simulink model "CloughExperimentGitHub"  (R2023a)
settings: Solver=ode45  StartTime=0.0  StopTime=t_end  FixedStep=1e-6  RelTol=relTol  AbsTol=absTol
values from neighbouring files (symbols this model uses):
  frame_rot = atan((L_beam*3/2)/(L_col/2))    [CloughExperiment.m]
  g = 9.80665    [CloughExperiment.m]    (also in Example1_CBReduction.m; GitHubVersion.m)
  gao = 1/4*chang    (= 0.3048)    [CloughExperiment.m]
  L_beam = 4*length_Convert    (= 1.2192)    [CloughExperiment.m]
  L_inplane = 6*length_Convert    (= 1.8288)    [CloughExperiment.m]
undefined symbols (not defined in the file or in its folder): aa3a, d5ee, X, Y, Z
libraries: sm_lib x165, slrealtimeloglib x29, nesl_utility x26, OxDynamicsContact x4, sharedtransform x1
(part 2 of 2)

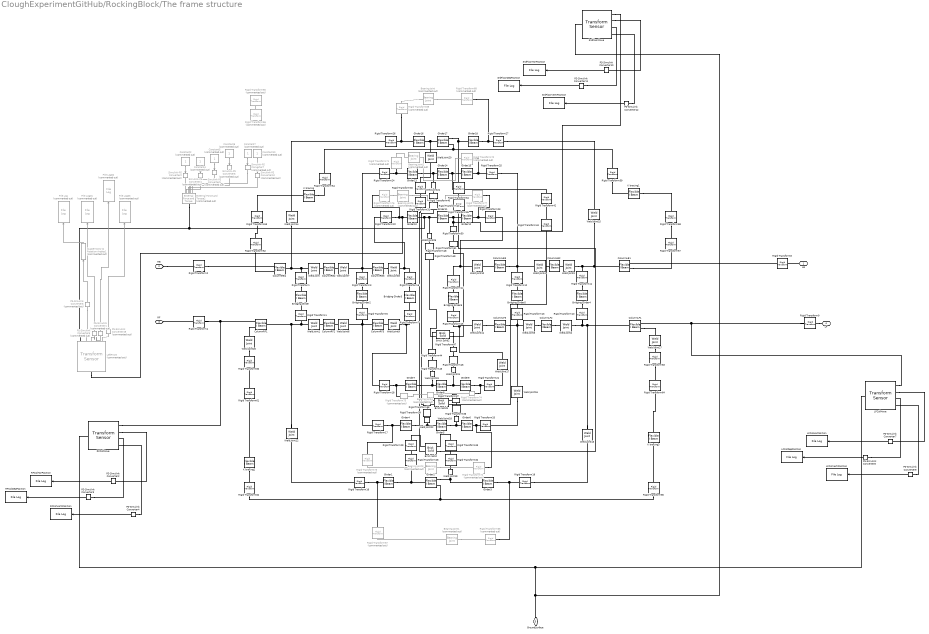
== system CloughExperimentGitHub/RockingBlock/The frame structure ==
  " LeftFront" : sm_lib/Frames and Transforms/Transform Sensor  Commented=on  MeasurementFrame=Base  RotationSequence=XYX  SenseAngle=off  SenseAxis=off  SenseQ=on  SenseR=off  SenseRotationSequence=off  SenseOmegaX=off  SenseOmegaY=off  SenseOmegaZ=off  SenseQDot=off  SenseRDot=off  SenseRotationSequenceDot=off  SenseAlphaX=off  SenseAlphaY=off  SenseAlphaZ=off  SenseQDDot=off  SenseRDDot=off  SenseX=on  SenseY=on  SenseZ=on  SenseRad=off  SenseAzim=off  SenseDist=off  SenseInc=off  SenseXDot=off  SenseYDot=off  SenseZDot=off  SenseRadDot=off  SenseAzimDot=off  SenseDistDot=off  SenseIncDot=off  SenseXDDot=off  SenseYDDot=off  SenseZDDot=off  SenseRadDDot=off  SenseAzimDDot=off  SenseDistDDot=off  SenseIncDDot=off
  3rdFloorDepPosition : slrealtimeloglib/File Log  decimation=200  inputProcessing=Elements as channels (sample based)
  3rdFloorHorPosition : slrealtimeloglib/File Log  decimation=200  inputProcessing=Elements as channels (sample based)
  3rdFloorMove : sm_lib/Frames and Transforms/Transform Sensor  MeasurementFrame=Base  RotationSequence=XYX  SenseAngle=off  SenseAxis=off  SenseQ=off  SenseR=off  SenseRotationSequence=off  SenseOmegaX=off  SenseOmegaY=off  SenseOmegaZ=off  SenseQDot=off  SenseRDot=off  SenseRotationSequenceDot=off  SenseAlphaX=off  SenseAlphaY=off  SenseAlphaZ=off  SenseQDDot=off  SenseRDDot=off  SenseX=on  SenseY=on  SenseZ=on  SenseRad=off  SenseAzim=off  SenseDist=off  SenseInc=off  SenseXDot=off  SenseYDot=off  SenseZDot=off  SenseRadDot=off  SenseAzimDot=off  SenseDistDot=off  SenseIncDot=off  SenseXDDot=off  SenseYDDot=off  SenseZDDot=off  SenseRadDDot=off  SenseAzimDDot=off  SenseDistDDot=off  SenseIncDDot=off
  3rdFloorVertiPosition : slrealtimeloglib/File Log  decimation=200  inputProcessing=Elements as channels (sample based)
  Bearing Joint{,1..5} (6 alike) : sm_lib/Joints/Bearing Joint  Commented=on  JointMode=Normal  SenseConstraintForce=off  SenseConstraintForceX=off  SenseConstraintForceY=off  SenseConstraintForceZ=off  SenseConstraintTorque=off  SenseConstraintTorqueX=off  SenseConstraintTorqueY=off  SenseConstraintTorqueZ=off  SenseTotalForce=off  SenseTotalForceX=off  SenseTotalForceY=off  SenseTotalForceZ=off  SenseTotalTorque=off  SenseTotalTorqueX=off  SenseTotalTorqueY=off  SenseTotalTorqueZ=off  CompositeWrenchDir=FollowerOnBase  CompositeWrenchFrame=BaseFrame  PzEquilibriumPosition=0  PzEquilibriumPositionUnits=m  PzSpringStiffness=0  PzSpringStiffnessUnits=N/m  PzDampingCoefficient=0  PzDampingCoefficientUnits=N/(m/s)  PzTorqueActuationMode=NoTorque  PzMotionActuationMode=ComputedMotion  PzSensePosition=off  PzSenseVelocity=off  PzSenseAcceleration=off  PzSenseTorqueForce=off  PzSenseLowerLimitTorqueForce=off  PzSenseUpperLimitTorqueForce=off  PzLowerLimitSpecify=off  PzLowerLimitBound=-1  PzLowerLimitBoundUnits=m  PzLowerLimitStiffness=1e6  PzLowerLimitStiffnessUnits=N/m  PzLowerLimitDamping=1e3  PzLowerLimitDampingUnits=N/(m/s)  PzLowerLimitTransitionRegionWidth=1e-4  PzLowerLimitTransitionRegionWidthUnits=m  PzUpperLimitSpecify=off  PzUpperLimitBound=1  PzUpperLimitBoundUnits=m  PzUpperLimitStiffness=1e6  PzUpperLimitStiffnessUnits=N/m  PzUpperLimitDamping=1e3  PzUpperLimitDampingUnits=N/(m/s)  PzUpperLimitTransitionRegionWidth=1e-4  PzUpperLimitTransitionRegionWidthUnits=m  PzPositionTargetSpecify=off  PzPositionTargetPriority=High  PzPositionTargetValue=0  PzPositionTargetValueUnits=m  PzVelocityTargetSpecify=off  PzVelocityTargetPriority=High  PzVelocityTargetValue=0  PzVelocityTargetValueUnits=m/s  RxEquilibriumPosition=0  RxEquilibriumPositionUnits=deg  RxSpringStiffness=0  RxSpringStiffnessUnits=N*m/deg  RxDampingCoefficient=0  RxDampingCoefficientUnits=N*m/(deg/s)  RxTorqueActuationMode=NoTorque  RxMotionActuationMode=ComputedMotion  RxSensePosition=off  RxSenseVelocity=off  RxSenseAcceleration=off  RxSenseTorqueForce=off  RxSenseLowerLimitTorqueForce=off  RxSenseUpperLimitTorqueForce=off  RxLowerLimitSpecify=off  RxLowerLimitBound=-90  RxLowerLimitBoundUnits=deg  RxLowerLimitStiffness=1e4  RxLowerLimitStiffnessUnits=N*m/deg  RxLowerLimitDamping=10  RxLowerLimitDampingUnits=N*m/(deg/s)  RxLowerLimitTransitionRegionWidth=0.1  RxLowerLimitTransitionRegionWidthUnits=deg  RxUpperLimitSpecify=off  RxUpperLimitBound=90  RxUpperLimitBoundUnits=deg  RxUpperLimitStiffness=1e4  RxUpperLimitStiffnessUnits=N*m/deg  RxUpperLimitDamping=10  RxUpperLimitDampingUnits=N*m/(deg/s)  RxUpperLimitTransitionRegionWidth=0.1  RxUpperLimitTransitionRegionWidthUnits=deg  RxPositionTargetSpecify=off  RxPositionTargetPriority=High  RxPositionTargetValue=0  RxPositionTargetValueUnits=deg  RxVelocityTargetSpecify=off  RxVelocityTargetPriority=High  RxVelocityTargetValue=0  RxVelocityTargetValueUnits=deg/s  RyEquilibriumPosition=0  RyEquilibriumPositionUnits=deg  RySpringStiffness=0  RySpringStiffnessUnits=N*m/deg  RyDampingCoefficient=0  RyDampingCoefficientUnits=N*m/(deg/s)  RyTorqueActuationMode=NoTorque  RyMotionActuationMode=ComputedMotion  RySensePosition=off  RySenseVelocity=off  RySenseAcceleration=off  RySenseTorqueForce=off  RySenseLowerLimitTorqueForce=off  RySenseUpperLimitTorqueForce=off  RyLowerLimitSpecify=off  RyLowerLimitBound=-90  RyLowerLimitBoundUnits=deg  RyLowerLimitStiffness=1e4  RyLowerLimitStiffnessUnits=N*m/deg  RyLowerLimitDamping=10  RyLowerLimitDampingUnits=N*m/(deg/s)  RyLowerLimitTransitionRegionWidth=0.1  RyLowerLimitTransitionRegionWidthUnits=deg  RyUpperLimitSpecify=off  RyUpperLimitBound=90  RyUpperLimitBoundUnits=deg  RyUpperLimitStiffness=1e4  RyUpperLimitStiffnessUnits=N*m/deg  RyUpperLimitDamping=10  RyUpperLimitDampingUnits=N*m/(deg/s)  RyUpperLimitTransitionRegionWidth=0.1  RyUpperLimitTransitionRegionWidthUnits=deg  RyPositionTargetSpecify=off  RyPositionTargetPriority=High  RyPositionTargetValue=0  RyPositionTargetValueUnits=deg  RyVelocityTargetSpecify=off  RyVelocityTargetPriority=High  RyVelocityTargetValue=0  RyVelocityTargetValueUnits=deg/s  RzEquilibriumPosition=0  RzEquilibriumPositionUnits=deg  RzSpringStiffness=0  RzSpringStiffnessUnits=N*m/deg  RzDampingCoefficient=0  RzDampingCoefficientUnits=N*m/(deg/s)  RzTorqueActuationMode=NoTorque  RzMotionActuationMode=ComputedMotion  RzSensePosition=off  RzSenseVelocity=off  RzSenseAcceleration=off  RzSenseTorqueForce=off  RzSenseLowerLimitTorqueForce=off  RzSenseUpperLimitTorqueForce=off  RzLowerLimitSpecify=off  RzLowerLimitBound=-90  RzLowerLimitBoundUnits=deg  RzLowerLimitStiffness=1e4  RzLowerLimitStiffnessUnits=N*m/deg  RzLowerLimitDamping=10  RzLowerLimitDampingUnits=N*m/(deg/s)  RzLowerLimitTransitionRegionWidth=0.1  RzLowerLimitTransitionRegionWidthUnits=deg  RzUpperLimitSpecify=off  RzUpperLimitBound=90  RzUpperLimitBoundUnits=deg  RzUpperLimitStiffness=1e4  RzUpperLimitStiffnessUnits=N*m/deg  RzUpperLimitDamping=10  RzUpperLimitDampingUnits=N*m/(deg/s)  RzUpperLimitTransitionRegionWidth=0.1  RzUpperLimitTransitionRegionWidthUnits=deg  RzPositionTargetSpecify=off  RzPositionTargetPriority=High  RzPositionTargetValue=0  RzPositionTargetValueUnits=deg  RzVelocityTargetSpecify=off  RzVelocityTargetPriority=High  RzVelocityTargetValue=0  RzVelocityTargetValueUnits=deg/s
  Brick Solid : sm_lib/Body Elements/Brick Solid  GraphicAmbientColor=[0.15 0.15 0.15 1.0]  BasedOnType=Density  BrickDimensions=[L_beam L_inplane gao]  BrickDimensionsUnits=m  CenterOfMass=[0 0 0]  CenterOfMassUnits=m  GraphicDiffuseColor=[0.5 0.5 0.5]  Density=rho_dw  DensityUnits=kg/m^3  DoExposeReferenceFrame=off  GraphicEmissiveColor=[0.0 0.0 0.0 1.0]  ExportEntireGeometry=off  SerializedFrames=<Frames><Frame><Id>Frame1</Id><Value><Name>F1</Name><Origin><Source>GeometricFeature</Source><FeatureName>-x +y -z point</FeatureName></Origin><PrimaryAxis><DefinedDirection>+Z</DefinedDirection><Source>ReferenceFrame</Source><SourceDirection>+Z</SourceDirection><FeatureName></FeatureName></PrimaryAxis><SecondaryAxis><DefinedDirection>+X</DefinedDirection><Source>ReferenceFrame</Source><SourceDirection>+X</SourceDirection><FeatureName></FeatureName></SecondaryAxis></Value></Frame><Frame><Id>Frame2</Id><Value><Name>F2</Name><Origin><Source>GeometricFeature</Source><FeatureName>+x +y -z point</FeatureName></Origin><PrimaryAxis><DefinedDirection>+Z</DefinedDirection><Source>ReferenceFrame</Source><SourceDirection>+Z</SourceDirection><FeatureName></FeatureName></PrimaryAxis><SecondaryAxis><DefinedDirection>+X</DefinedDirection><Source>ReferenceFrame</Source><SourceDirection>+X</SourceDirection><FeatureName></FeatureName></SecondaryAxis></Value></Frame><Frame><Id>Frame3</Id><Value><Name>F3</Name><Origin><Source>GeometricFeature</Source><FeatureName>-x -y -z point</FeatureName></Origin><PrimaryAxis><DefinedDirection>+Z</DefinedDirection><Source>ReferenceFrame</Source><SourceDirection>+Z</SourceDirection><FeatureName></FeatureName></PrimaryAxis><SecondaryAxis><DefinedDirection>+X</DefinedDirection><Source>ReferenceFrame</Source><SourceDirection>+X</SourceDirection><FeatureName></FeatureName></SecondaryAxis></Value></Frame><Frame><Id>Frame4</Id><Value><Name>F4</Name><Origin><Source>GeometricFeature</Source><FeatureName>+x -y -z point</FeatureName></Origin><PrimaryAxis><DefinedDirection>+Z</DefinedDirection><Source>ReferenceFrame</Source><SourceDirection>+Z</SourceDirection><FeatureName></FeatureName></PrimaryAxis><SecondaryAxis><DefinedDirection>+X</DefinedDirection><Source>ReferenceFrame</Source><SourceDirection>+X</SourceDirection><FeatureName></FeatureName></SecondaryAxis></Value></Frame></Frames>  MarkerShape=Sphere  MarkerSize=10  GraphicType=FromGeometry  InertiaType=CalculateFromGeometry  Mass=1  MassUnits=kg  MomentsOfInertia=[1 1 1]  MomentsOfInertiaUnits=kg*m^2  GraphicOpacity=1.0  ProductsOfInertia=[0 0 0]  ProductsOfInertiaUnits=kg*m^2  GraphicShininess=75  GraphicSpecularColor=[0.5 0.5 0.5 1.0]  GraphicVisPropType=SimpleVisualProperties
  Brick Solid1 : sm_lib/Body Elements/Brick Solid  GraphicAmbientColor=[0.15 0.15 0.15 1.0]  BasedOnType=Density  BrickDimensions=[L_beam L_inplane gao]  BrickDimensionsUnits=m  CenterOfMass=[0 0 0]  CenterOfMassUnits=m  GraphicDiffuseColor=[0.5 0.5 0.5]  Density=rho_dw  DensityUnits=kg/m^3  DoExposeReferenceFrame=off  GraphicEmissiveColor=[0.0 0.0 0.0 1.0]  ExportEntireGeometry=off  SerializedFrames=<Frames><Frame><Id>Frame1</Id><Value><Name>F1</Name><Origin><Source>GeometricFeature</Source><FeatureName>-x +y -z point</FeatureName></Origin><PrimaryAxis><DefinedDirection>+Z</DefinedDirection><Source>ReferenceFrame</Source><SourceDirection>+Z</SourceDirection><FeatureName></FeatureName></PrimaryAxis><SecondaryAxis><DefinedDirection>+X</DefinedDirection><Source>ReferenceFrame</Source><SourceDirection>+X</SourceDirection><FeatureName></FeatureName></SecondaryAxis></Value></Frame><Frame><Id>Frame2</Id><Value><Name>F2</Name><Origin><Source>GeometricFeature</Source><FeatureName>+x +y -z point</FeatureName></Origin><PrimaryAxis><DefinedDirection>+Z</DefinedDirection><Source>ReferenceFrame</Source><SourceDirection>+Z</SourceDirection><FeatureName></FeatureName></PrimaryAxis><SecondaryAxis><DefinedDirection>+X</DefinedDirection><Source>ReferenceFrame</Source><SourceDirection>+X</SourceDirection><FeatureName></FeatureName></SecondaryAxis></Value></Frame><Frame><Id>Frame3</Id><Value><Name>F3</Name><Origin><Source>GeometricFeature</Source><FeatureName>-x -y -z point</FeatureName></Origin><PrimaryAxis><DefinedDirection>+Z</DefinedDirection><Source>ReferenceFrame</Source><SourceDirection>+Z</SourceDirection><FeatureName></FeatureName></PrimaryAxis><SecondaryAxis><DefinedDirection>+X</DefinedDirection><Source>ReferenceFrame</Source><SourceDirection>+X</SourceDirection><FeatureName></FeatureName></SecondaryAxis></Value></Frame><Frame><Id>Frame4</Id><Value><Name>F4</Name><Origin><Source>GeometricFeature</Source><FeatureName>+x -y -z point</FeatureName></Origin><PrimaryAxis><DefinedDirection>+Z</DefinedDirection><Source>ReferenceFrame</Source><SourceDirection>+Z</SourceDirection><FeatureName></FeatureName></PrimaryAxis><SecondaryAxis><DefinedDirection>+X</DefinedDirection><Source>ReferenceFrame</Source><SourceDirection>+X</SourceDirection><FeatureName></FeatureName></SecondaryAxis></Value></Frame></Frames>  MarkerShape=Sphere  MarkerSize=10  GraphicType=FromGeometry  InertiaType=CalculateFromGeometry  Mass=1  MassUnits=kg  MomentsOfInertia=[1 1 1]  MomentsOfInertiaUnits=kg*m^2  GraphicOpacity=1.0  ProductsOfInertia=[0 0 0]  ProductsOfInertiaUnits=kg*m^2  GraphicShininess=75  GraphicSpecularColor=[0.5 0.5 0.5 1.0]  GraphicVisPropType=SimpleVisualProperties
  Brick Solid2 : sm_lib/Body Elements/Brick Solid  GraphicAmbientColor=[0.15 0.15 0.15 1.0]  BasedOnType=Density  BrickDimensions=[L_beam L_inplane gao]  BrickDimensionsUnits=m  CenterOfMass=[0 0 0]  CenterOfMassUnits=m  GraphicDiffuseColor=[0.5 0.5 0.5]  Density=rho_dw  DensityUnits=kg/m^3  DoExposeReferenceFrame=off  GraphicEmissiveColor=[0.0 0.0 0.0 1.0]  ExportEntireGeometry=off  SerializedFrames=<Frames><Frame><Id>Frame1</Id><Value><Name>F1</Name><Origin><Source>GeometricFeature</Source><FeatureName>-x +y -z point</FeatureName></Origin><PrimaryAxis><DefinedDirection>+Z</DefinedDirection><Source>ReferenceFrame</Source><SourceDirection>+Z</SourceDirection><FeatureName></FeatureName></PrimaryAxis><SecondaryAxis><DefinedDirection>+X</DefinedDirection><Source>ReferenceFrame</Source><SourceDirection>+X</SourceDirection><FeatureName></FeatureName></SecondaryAxis></Value></Frame><Frame><Id>Frame2</Id><Value><Name>F2</Name><Origin><Source>GeometricFeature</Source><FeatureName>+x +y -z point</FeatureName></Origin><PrimaryAxis><DefinedDirection>+Z</DefinedDirection><Source>ReferenceFrame</Source><SourceDirection>+Z</SourceDirection><FeatureName></FeatureName></PrimaryAxis><SecondaryAxis><DefinedDirection>+X</DefinedDirection><Source>ReferenceFrame</Source><SourceDirection>+X</SourceDirection><FeatureName></FeatureName></SecondaryAxis></Value></Frame><Frame><Id>Frame3</Id><Value><Name>F3</Name><Origin><Source>GeometricFeature</Source><FeatureName>-x -y -z point</FeatureName></Origin><PrimaryAxis><DefinedDirection>+Z</DefinedDirection><Source>ReferenceFrame</Source><SourceDirection>+Z</SourceDirection><FeatureName></FeatureName></PrimaryAxis><SecondaryAxis><DefinedDirection>+X</DefinedDirection><Source>ReferenceFrame</Source><SourceDirection>+X</SourceDirection><FeatureName></FeatureName></SecondaryAxis></Value></Frame><Frame><Id>Frame4</Id><Value><Name>F4</Name><Origin><Source>GeometricFeature</Source><FeatureName>+x -y -z point</FeatureName></Origin><PrimaryAxis><DefinedDirection>+Z</DefinedDirection><Source>ReferenceFrame</Source><SourceDirection>+Z</SourceDirection><FeatureName></FeatureName></PrimaryAxis><SecondaryAxis><DefinedDirection>+X</DefinedDirection><Source>ReferenceFrame</Source><SourceDirection>+X</SourceDirection><FeatureName></FeatureName></SecondaryAxis></Value></Frame></Frames>  MarkerShape=Sphere  MarkerSize=10  GraphicType=FromGeometry  InertiaType=CalculateFromGeometry  Mass=1  MassUnits=kg  MomentsOfInertia=[1 1 1]  MomentsOfInertiaUnits=kg*m^2  GraphicOpacity=1.0  ProductsOfInertia=[0 0 0]  ProductsOfInertiaUnits=kg*m^2  GraphicShininess=75  GraphicSpecularColor=[0.5 0.5 0.5 1.0]  GraphicVisPropType=SimpleVisualProperties
  Bridging Girder{,2..6} (6 alike) : sm_lib/Body Elements/Flexible Bodies/Beams/Flexible I Beam  GraphicAmbientColor=[0.15 0.15 0.15 1.0]  AxialRigidity=1  AxialRigidityUnits=Pa*m^2  BendingCentroid=[0 0]  BendingCentroidUnits=m  FlexuralRigidity=[1 1]  FlexuralRigidityUnits=Pa*m^4  BottomFlangeThickness=beam_ft  BottomFlangeThicknessUnits=m  BottomFlangeWidth=beam_fw  BottomFlangeWidthUnits=m  CenterOfMass=[0 0]  CenterOfMassUnits=m  GraphicDiffuseColor=[0.5 0.5 0.5]  CrossFlexuralRigidity=0  CrossFlexuralRigidityUnits=Pa*m^4  SerializedFrames=<Frames/>  DampingType=UniformModal  Density=rho_steel  DensityUnits=kg/m^3  DoExposeZmaxFrame=on  DoExposeZminFrame=on  GraphicEmissiveColor=[0.0 0.0 0.0 1.0]  GeometricCentroid=[0 0]  GeometricCentroidUnits=m  GraphicType=FromGeometry  EndToEndHeight=beam_depth  EndToEndHeightUnits=m  Length=L_inplane  LengthUnits=m  MassMomentOfInertiaDensity=[1 1]  MassMomentOfInertiaDensityUnits=kg*m  MassPerUnitLength=1  MassPerUnitLengthUnits=kg/m  MassProductOfInertiaDensity=0  MassProductOfInertiaDensityUnits=kg*m  ModuliType=YoungsPoissons  NumElements=1  NumRetainedModes=1  GraphicOpacity=1.0  PoissonsRatio=p_steel  ReductionType=None  ShearCenter=[0 0]  ShearCenterUnits=m  ShearModulus=26  ShearModulusUnits=GPa  GraphicShininess=75  GraphicSpecularColor=[0.5 0.5 0.5 1.0]  StiffnessAndInertiaType=CalculateFromGeometry  TopFlangeThickness=beam_ft  TopFlangeThicknessUnits=m  TopFlangeWidth=beam_fw  TopFlangeWidthUnits=m  TorsionalRigidity=1  TorsionalRigidityUnits=Pa*m^4  GraphicVisPropType=SimpleVisualProperties  WebThickness=beam_wt  WebThicknessUnits=m  YoungsModulus=E_steel  YoungsModulusUnits=Pa  ProportionalDampingAlpha=0  ProportionalDampingAlphaUnits=1/s  ProportionalDampingBeta=0.001  ProportionalDampingBetaUnits=s  UniformModalDampingRatio=uni_dr
  ColumnLB1 : sm_lib/Body Elements/Flexible Bodies/Beams/Flexible I Beam  GraphicAmbientColor=[0.15 0.15 0.15 1.0]  AxialRigidity=1  AxialRigidityUnits=Pa*m^2  BendingCentroid=[0 0]  BendingCentroidUnits=m  FlexuralRigidity=[1 1]  FlexuralRigidityUnits=Pa*m^4  BottomFlangeThickness=col_ft  BottomFlangeThicknessUnits=m  BottomFlangeWidth=col_fw  BottomFlangeWidthUnits=m  CenterOfMass=[0 0]  CenterOfMassUnits=m  GraphicDiffuseColor=[0.5 0.5 0.5]  CrossFlexuralRigidity=0  CrossFlexuralRigidityUnits=Pa*m^4  SerializedFrames=<Frames><Frame><Id>Frame1</Id><Value><Name>Middle</Name><Origin><Source>ReferenceFrame</Source><FeatureName></FeatureName></Origin><PrimaryAxis><DefinedDirection>+Z</DefinedDirection><Source>ReferenceFrame</Source><SourceDirection>+Z</SourceDirection><FeatureName></FeatureName></PrimaryAxis><SecondaryAxis><DefinedDirection>+X</DefinedDirection><Source>ReferenceFrame</Source><SourceDirection>+X</SourceDirection><FeatureName></FeatureName></SecondaryAxis></Value></Frame></Frames>  DampingType=UniformModal  Density=rho_steel  DensityUnits=kg/m^3  DoExposeZmaxFrame=on  DoExposeZminFrame=on  GraphicEmissiveColor=[0.0 0.0 0.0 1.0]  GeometricCentroid=[0 0]  GeometricCentroidUnits=m  GraphicType=FromGeometry  EndToEndHeight=col_depth  EndToEndHeightUnits=m  Length=L_col  LengthUnits=m  MassMomentOfInertiaDensity=[1 1]  MassMomentOfInertiaDensityUnits=kg*m  MassPerUnitLength=1  MassPerUnitLengthUnits=kg/m  MassProductOfInertiaDensity=0  MassProductOfInertiaDensityUnits=kg*m  ModuliType=YoungsPoissons  NumElements=2  NumRetainedModes=1  GraphicOpacity=1.0  PoissonsRatio=p_steel  ReductionType=None  ShearCenter=[0 0]  ShearCenterUnits=m  ShearModulus=26  ShearModulusUnits=GPa  GraphicShininess=75  GraphicSpecularColor=[0.5 0.5 0.5 1.0]  StiffnessAndInertiaType=CalculateFromGeometry  TopFlangeThickness=col_ft  TopFlangeThicknessUnits=m  TopFlangeWidth=col_fw  TopFlangeWidthUnits=m  TorsionalRigidity=1  TorsionalRigidityUnits=Pa*m^4  GraphicVisPropType=SimpleVisualProperties  WebThickness=col_wt  WebThicknessUnits=m  YoungsModulus=E_steel  YoungsModulusUnits=Pa  ProportionalDampingAlpha=0  ProportionalDampingAlphaUnits=1/s  ProportionalDampingBeta=0.001  ProportionalDampingBetaUnits=s  UniformModalDampingRatio=uni_dr
  ColumnLB2 : sm_lib/Body Elements/Flexible Bodies/Beams/Flexible I Beam  GraphicAmbientColor=[0.15 0.15 0.15 1.0]  AxialRigidity=1  AxialRigidityUnits=Pa*m^2  BendingCentroid=[0 0]  BendingCentroidUnits=m  FlexuralRigidity=[1 1]  FlexuralRigidityUnits=Pa*m^4  BottomFlangeThickness=col_ft  BottomFlangeThicknessUnits=m  BottomFlangeWidth=col_fw  BottomFlangeWidthUnits=m  CenterOfMass=[0 0]  CenterOfMassUnits=m  GraphicDiffuseColor=[0.5 0.5 0.5]  CrossFlexuralRigidity=0  CrossFlexuralRigidityUnits=Pa*m^4  SerializedFrames=<Frames/>  DampingType=UniformModal  Density=rho_steel  DensityUnits=kg/m^3  DoExposeZmaxFrame=on  DoExposeZminFrame=on  GraphicEmissiveColor=[0.0 0.0 0.0 1.0]  GeometricCentroid=[0 0]  GeometricCentroidUnits=m  GraphicType=FromGeometry  EndToEndHeight=col_depth  EndToEndHeightUnits=m  Length=L_col2  LengthUnits=m  MassMomentOfInertiaDensity=[1 1]  MassMomentOfInertiaDensityUnits=kg*m  MassPerUnitLength=1  MassPerUnitLengthUnits=kg/m  MassProductOfInertiaDensity=0  MassProductOfInertiaDensityUnits=kg*m  ModuliType=YoungsPoissons  NumElements=1  NumRetainedModes=1  GraphicOpacity=1.0  PoissonsRatio=p_steel  ReductionType=None  ShearCenter=[0 0]  ShearCenterUnits=m  ShearModulus=26  ShearModulusUnits=GPa  GraphicShininess=75  GraphicSpecularColor=[0.5 0.5 0.5 1.0]  StiffnessAndInertiaType=CalculateFromGeometry  TopFlangeThickness=col_ft  TopFlangeThicknessUnits=m  TopFlangeWidth=col_fw  TopFlangeWidthUnits=m  TorsionalRigidity=1  TorsionalRigidityUnits=Pa*m^4  GraphicVisPropType=SimpleVisualProperties  WebThickness=col_wt  WebThicknessUnits=m  YoungsModulus=E_steel  YoungsModulusUnits=Pa  ProportionalDampingAlpha=0  ProportionalDampingAlphaUnits=1/s  ProportionalDampingBeta=0.001  ProportionalDampingBetaUnits=s  UniformModalDampingRatio=uni_dr
  ColumnLB3 : sm_lib/Body Elements/Flexible Bodies/Beams/Flexible I Beam  GraphicAmbientColor=[0.15 0.15 0.15 1.0]  AxialRigidity=1  AxialRigidityUnits=Pa*m^2  BendingCentroid=[0 0]  BendingCentroidUnits=m  FlexuralRigidity=[1 1]  FlexuralRigidityUnits=Pa*m^4  BottomFlangeThickness=col_ft  BottomFlangeThicknessUnits=m  BottomFlangeWidth=col_fw  BottomFlangeWidthUnits=m  CenterOfMass=[0 0]  CenterOfMassUnits=m  GraphicDiffuseColor=[0.5 0.5 0.5]  CrossFlexuralRigidity=0  CrossFlexuralRigidityUnits=Pa*m^4  SerializedFrames=<Frames/>  DampingType=UniformModal  Density=rho_steel  DensityUnits=kg/m^3  DoExposeZmaxFrame=on  DoExposeZminFrame=on  GraphicEmissiveColor=[0.0 0.0 0.0 1.0]  GeometricCentroid=[0 0]  GeometricCentroidUnits=m  GraphicType=FromGeometry  EndToEndHeight=col_depth  EndToEndHeightUnits=m  Length=L_col3  LengthUnits=m  MassMomentOfInertiaDensity=[1 1]  MassMomentOfInertiaDensityUnits=kg*m  MassPerUnitLength=1  MassPerUnitLengthUnits=kg/m  MassProductOfInertiaDensity=0  MassProductOfInertiaDensityUnits=kg*m  ModuliType=YoungsPoissons  NumElements=1  NumRetainedModes=1  GraphicOpacity=1.0  PoissonsRatio=p_steel  ReductionType=None  ShearCenter=[0 0]  ShearCenterUnits=m  ShearModulus=26  ShearModulusUnits=GPa  GraphicShininess=75  GraphicSpecularColor=[0.5 0.5 0.5 1.0]  StiffnessAndInertiaType=CalculateFromGeometry  TopFlangeThickness=col_ft  TopFlangeThicknessUnits=m  TopFlangeWidth=col_fw  TopFlangeWidthUnits=m  TorsionalRigidity=1  TorsionalRigidityUnits=Pa*m^4  GraphicVisPropType=SimpleVisualProperties  WebThickness=col_wt  WebThicknessUnits=m  YoungsModulus=E_steel  YoungsModulusUnits=Pa  ProportionalDampingAlpha=0  ProportionalDampingAlphaUnits=1/s  ProportionalDampingBeta=0.001  ProportionalDampingBetaUnits=s  UniformModalDampingRatio=uni_dr
  ColumnLF1 : sm_lib/Body Elements/Flexible Bodies/Beams/Flexible I Beam  GraphicAmbientColor=[0.15 0.15 0.15 1.0]  AxialRigidity=1  AxialRigidityUnits=Pa*m^2  BendingCentroid=[0 0]  BendingCentroidUnits=m  FlexuralRigidity=[1 1]  FlexuralRigidityUnits=Pa*m^4  BottomFlangeThickness=col_ft  BottomFlangeThicknessUnits=m  BottomFlangeWidth=col_fw  BottomFlangeWidthUnits=m  CenterOfMass=[0 0]  CenterOfMassUnits=m  GraphicDiffuseColor=[0.5 0.5 0.5]  CrossFlexuralRigidity=0  CrossFlexuralRigidityUnits=Pa*m^4  SerializedFrames=<Frames><Frame><Id>Frame1</Id><Value><Name>Middle</Name><Origin><Source>ReferenceFrame</Source><FeatureName></FeatureName></Origin><PrimaryAxis><DefinedDirection>+Z</DefinedDirection><Source>ReferenceFrame</Source><SourceDirection>+Z</SourceDirection><FeatureName></FeatureName></PrimaryAxis><SecondaryAxis><DefinedDirection>+X</DefinedDirection><Source>ReferenceFrame</Source><SourceDirection>+X</SourceDirection><FeatureName></FeatureName></SecondaryAxis></Value></Frame></Frames>  DampingType=UniformModal  Density=rho_steel  DensityUnits=kg/m^3  DoExposeZmaxFrame=on  DoExposeZminFrame=on  GraphicEmissiveColor=[0.0 0.0 0.0 1.0]  GeometricCentroid=[0 0]  GeometricCentroidUnits=m  GraphicType=FromGeometry  EndToEndHeight=col_depth  EndToEndHeightUnits=m  Length=L_col  LengthUnits=m  MassMomentOfInertiaDensity=[1 1]  MassMomentOfInertiaDensityUnits=kg*m  MassPerUnitLength=1  MassPerUnitLengthUnits=kg/m  MassProductOfInertiaDensity=0  MassProductOfInertiaDensityUnits=kg*m  ModuliType=YoungsPoissons  NumElements=2  NumRetainedModes=1  GraphicOpacity=1.0  PoissonsRatio=p_steel  ReductionType=None  ShearCenter=[0 0]  ShearCenterUnits=m  ShearModulus=26  ShearModulusUnits=GPa  GraphicShininess=75  GraphicSpecularColor=[0.5 0.5 0.5 1.0]  StiffnessAndInertiaType=CalculateFromGeometry  TopFlangeThickness=col_ft  TopFlangeThicknessUnits=m  TopFlangeWidth=col_fw  TopFlangeWidthUnits=m  TorsionalRigidity=1  TorsionalRigidityUnits=Pa*m^4  GraphicVisPropType=SimpleVisualProperties  WebThickness=col_wt  WebThicknessUnits=m  YoungsModulus=E_steel  YoungsModulusUnits=Pa  ProportionalDampingAlpha=0  ProportionalDampingAlphaUnits=1/s  ProportionalDampingBeta=0.001  ProportionalDampingBetaUnits=s  UniformModalDampingRatio=uni_dr
  ColumnLF2 : sm_lib/Body Elements/Flexible Bodies/Beams/Flexible I Beam  GraphicAmbientColor=[0.15 0.15 0.15 1.0]  AxialRigidity=1  AxialRigidityUnits=Pa*m^2  BendingCentroid=[0 0]  BendingCentroidUnits=m  FlexuralRigidity=[1 1]  FlexuralRigidityUnits=Pa*m^4  BottomFlangeThickness=col_ft  BottomFlangeThicknessUnits=m  BottomFlangeWidth=col_fw  BottomFlangeWidthUnits=m  CenterOfMass=[0 0]  CenterOfMassUnits=m  GraphicDiffuseColor=[0.5 0.5 0.5]  CrossFlexuralRigidity=0  CrossFlexuralRigidityUnits=Pa*m^4  SerializedFrames=<Frames/>  DampingType=UniformModal  Density=rho_steel  DensityUnits=kg/m^3  DoExposeZmaxFrame=on  DoExposeZminFrame=on  GraphicEmissiveColor=[0.0 0.0 0.0 1.0]  GeometricCentroid=[0 0]  GeometricCentroidUnits=m  GraphicType=FromGeometry  EndToEndHeight=col_depth  EndToEndHeightUnits=m  Length=L_col2  LengthUnits=m  MassMomentOfInertiaDensity=[1 1]  MassMomentOfInertiaDensityUnits=kg*m  MassPerUnitLength=1  MassPerUnitLengthUnits=kg/m  MassProductOfInertiaDensity=0  MassProductOfInertiaDensityUnits=kg*m  ModuliType=YoungsPoissons  NumElements=1  NumRetainedModes=1  GraphicOpacity=1.0  PoissonsRatio=p_steel  ReductionType=None  ShearCenter=[0 0]  ShearCenterUnits=m  ShearModulus=26  ShearModulusUnits=GPa  GraphicShininess=75  GraphicSpecularColor=[0.5 0.5 0.5 1.0]  StiffnessAndInertiaType=CalculateFromGeometry  TopFlangeThickness=col_ft  TopFlangeThicknessUnits=m  TopFlangeWidth=col_fw  TopFlangeWidthUnits=m  TorsionalRigidity=1  TorsionalRigidityUnits=Pa*m^4  GraphicVisPropType=SimpleVisualProperties  WebThickness=col_wt  WebThicknessUnits=m  YoungsModulus=E_steel  YoungsModulusUnits=Pa  ProportionalDampingAlpha=0  ProportionalDampingAlphaUnits=1/s  ProportionalDampingBeta=0.001  ProportionalDampingBetaUnits=s  UniformModalDampingRatio=uni_dr
  ColumnLF3 : sm_lib/Body Elements/Flexible Bodies/Beams/Flexible I Beam  GraphicAmbientColor=[0.15 0.15 0.15 1.0]  AxialRigidity=1  AxialRigidityUnits=Pa*m^2  BendingCentroid=[0 0]  BendingCentroidUnits=m  FlexuralRigidity=[1 1]  FlexuralRigidityUnits=Pa*m^4  BottomFlangeThickness=col_ft  BottomFlangeThicknessUnits=m  BottomFlangeWidth=col_fw  BottomFlangeWidthUnits=m  CenterOfMass=[0 0]  CenterOfMassUnits=m  GraphicDiffuseColor=[0.5 0.5 0.5]  CrossFlexuralRigidity=0  CrossFlexuralRigidityUnits=Pa*m^4  SerializedFrames=<Frames/>  DampingType=UniformModal  Density=rho_steel  DensityUnits=kg/m^3  DoExposeZmaxFrame=on  DoExposeZminFrame=on  GraphicEmissiveColor=[0.0 0.0 0.0 1.0]  GeometricCentroid=[0 0]  GeometricCentroidUnits=m  GraphicType=FromGeometry  EndToEndHeight=col_depth  EndToEndHeightUnits=m  Length=L_col3  LengthUnits=m  MassMomentOfInertiaDensity=[1 1]  MassMomentOfInertiaDensityUnits=kg*m  MassPerUnitLength=1  MassPerUnitLengthUnits=kg/m  MassProductOfInertiaDensity=0  MassProductOfInertiaDensityUnits=kg*m  ModuliType=YoungsPoissons  NumElements=1  NumRetainedModes=1  GraphicOpacity=1.0  PoissonsRatio=p_steel  ReductionType=None  ShearCenter=[0 0]  ShearCenterUnits=m  ShearModulus=26  ShearModulusUnits=GPa  GraphicShininess=75  GraphicSpecularColor=[0.5 0.5 0.5 1.0]  StiffnessAndInertiaType=CalculateFromGeometry  TopFlangeThickness=col_ft  TopFlangeThicknessUnits=m  TopFlangeWidth=col_fw  TopFlangeWidthUnits=m  TorsionalRigidity=1  TorsionalRigidityUnits=Pa*m^4  GraphicVisPropType=SimpleVisualProperties  WebThickness=col_wt  WebThicknessUnits=m  YoungsModulus=E_steel  YoungsModulusUnits=Pa  ProportionalDampingAlpha=0  ProportionalDampingAlphaUnits=1/s  ProportionalDampingBeta=0.001  ProportionalDampingBetaUnits=s  UniformModalDampingRatio=uni_dr
  ColumnRB1 : sm_lib/Body Elements/Flexible Bodies/Beams/Flexible I Beam  GraphicAmbientColor=[0.15 0.15 0.15 1.0]  AxialRigidity=1  AxialRigidityUnits=Pa*m^2  BendingCentroid=[0 0]  BendingCentroidUnits=m  FlexuralRigidity=[1 1]  FlexuralRigidityUnits=Pa*m^4  BottomFlangeThickness=col_ft  BottomFlangeThicknessUnits=m  BottomFlangeWidth=col_fw  BottomFlangeWidthUnits=m  CenterOfMass=[0 0]  CenterOfMassUnits=m  GraphicDiffuseColor=[0.5 0.5 0.5]  CrossFlexuralRigidity=0  CrossFlexuralRigidityUnits=Pa*m^4  SerializedFrames=<Frames><Frame><Id>Frame1</Id><Value><Name>Middle</Name><Origin><Source>ReferenceFrame</Source><FeatureName></FeatureName></Origin><PrimaryAxis><DefinedDirection>+Z</DefinedDirection><Source>ReferenceFrame</Source><SourceDirection>+Z</SourceDirection><FeatureName></FeatureName></PrimaryAxis><SecondaryAxis><DefinedDirection>+X</DefinedDirection><Source>ReferenceFrame</Source><SourceDirection>+X</SourceDirection><FeatureName></FeatureName></SecondaryAxis></Value></Frame></Frames>  DampingType=UniformModal  Density=rho_steel  DensityUnits=kg/m^3  DoExposeZmaxFrame=on  DoExposeZminFrame=on  GraphicEmissiveColor=[0.0 0.0 0.0 1.0]  GeometricCentroid=[0 0]  GeometricCentroidUnits=m  GraphicType=FromGeometry  EndToEndHeight=col_depth  EndToEndHeightUnits=m  Length=L_col  LengthUnits=m  MassMomentOfInertiaDensity=[1 1]  MassMomentOfInertiaDensityUnits=kg*m  MassPerUnitLength=1  MassPerUnitLengthUnits=kg/m  MassProductOfInertiaDensity=0  MassProductOfInertiaDensityUnits=kg*m  ModuliType=YoungsPoissons  NumElements=2  NumRetainedModes=1  GraphicOpacity=1.0  PoissonsRatio=p_steel  ReductionType=None  ShearCenter=[0 0]  ShearCenterUnits=m  ShearModulus=26  ShearModulusUnits=GPa  GraphicShininess=75  GraphicSpecularColor=[0.5 0.5 0.5 1.0]  StiffnessAndInertiaType=CalculateFromGeometry  TopFlangeThickness=col_ft  TopFlangeThicknessUnits=m  TopFlangeWidth=col_fw  TopFlangeWidthUnits=m  TorsionalRigidity=1  TorsionalRigidityUnits=Pa*m^4  GraphicVisPropType=SimpleVisualProperties  WebThickness=col_wt  WebThicknessUnits=m  YoungsModulus=E_steel  YoungsModulusUnits=Pa  ProportionalDampingAlpha=0  ProportionalDampingAlphaUnits=1/s  ProportionalDampingBeta=0.001  ProportionalDampingBetaUnits=s  UniformModalDampingRatio=uni_dr
  ColumnRB2 : sm_lib/Body Elements/Flexible Bodies/Beams/Flexible I Beam  GraphicAmbientColor=[0.15 0.15 0.15 1.0]  AxialRigidity=1  AxialRigidityUnits=Pa*m^2  BendingCentroid=[0 0]  BendingCentroidUnits=m  FlexuralRigidity=[1 1]  FlexuralRigidityUnits=Pa*m^4  BottomFlangeThickness=col_ft  BottomFlangeThicknessUnits=m  BottomFlangeWidth=col_fw  BottomFlangeWidthUnits=m  CenterOfMass=[0 0]  CenterOfMassUnits=m  GraphicDiffuseColor=[0.5 0.5 0.5]  CrossFlexuralRigidity=0  CrossFlexuralRigidityUnits=Pa*m^4  SerializedFrames=<Frames/>  DampingType=UniformModal  Density=rho_steel  DensityUnits=kg/m^3  DoExposeZmaxFrame=on  DoExposeZminFrame=on  GraphicEmissiveColor=[0.0 0.0 0.0 1.0]  GeometricCentroid=[0 0]  GeometricCentroidUnits=m  GraphicType=FromGeometry  EndToEndHeight=col_depth  EndToEndHeightUnits=m  Length=L_col2  LengthUnits=m  MassMomentOfInertiaDensity=[1 1]  MassMomentOfInertiaDensityUnits=kg*m  MassPerUnitLength=1  MassPerUnitLengthUnits=kg/m  MassProductOfInertiaDensity=0  MassProductOfInertiaDensityUnits=kg*m  ModuliType=YoungsPoissons  NumElements=1  NumRetainedModes=1  GraphicOpacity=1.0  PoissonsRatio=p_steel  ReductionType=None  ShearCenter=[0 0]  ShearCenterUnits=m  ShearModulus=26  ShearModulusUnits=GPa  GraphicShininess=75  GraphicSpecularColor=[0.5 0.5 0.5 1.0]  StiffnessAndInertiaType=CalculateFromGeometry  TopFlangeThickness=col_ft  TopFlangeThicknessUnits=m  TopFlangeWidth=col_fw  TopFlangeWidthUnits=m  TorsionalRigidity=1  TorsionalRigidityUnits=Pa*m^4  GraphicVisPropType=SimpleVisualProperties  WebThickness=col_wt  WebThicknessUnits=m  YoungsModulus=E_steel  YoungsModulusUnits=Pa  ProportionalDampingAlpha=0  ProportionalDampingAlphaUnits=1/s  ProportionalDampingBeta=0.001  ProportionalDampingBetaUnits=s  UniformModalDampingRatio=uni_dr
  ColumnRB3 : sm_lib/Body Elements/Flexible Bodies/Beams/Flexible I Beam  GraphicAmbientColor=[0.15 0.15 0.15 1.0]  AxialRigidity=1  AxialRigidityUnits=Pa*m^2  BendingCentroid=[0 0]  BendingCentroidUnits=m  FlexuralRigidity=[1 1]  FlexuralRigidityUnits=Pa*m^4  BottomFlangeThickness=col_ft  BottomFlangeThicknessUnits=m  BottomFlangeWidth=col_fw  BottomFlangeWidthUnits=m  CenterOfMass=[0 0]  CenterOfMassUnits=m  GraphicDiffuseColor=[0.5 0.5 0.5]  CrossFlexuralRigidity=0  CrossFlexuralRigidityUnits=Pa*m^4  SerializedFrames=<Frames/>  DampingType=UniformModal  Density=rho_steel  DensityUnits=kg/m^3  DoExposeZmaxFrame=on  DoExposeZminFrame=on  GraphicEmissiveColor=[0.0 0.0 0.0 1.0]  GeometricCentroid=[0 0]  GeometricCentroidUnits=m  GraphicType=FromGeometry  EndToEndHeight=col_depth  EndToEndHeightUnits=m  Length=L_col3  LengthUnits=m  MassMomentOfInertiaDensity=[1 1]  MassMomentOfInertiaDensityUnits=kg*m  MassPerUnitLength=1  MassPerUnitLengthUnits=kg/m  MassProductOfInertiaDensity=0  MassProductOfInertiaDensityUnits=kg*m  ModuliType=YoungsPoissons  NumElements=1  NumRetainedModes=1  GraphicOpacity=1.0  PoissonsRatio=p_steel  ReductionType=None  ShearCenter=[0 0]  ShearCenterUnits=m  ShearModulus=26  ShearModulusUnits=GPa  GraphicShininess=75  GraphicSpecularColor=[0.5 0.5 0.5 1.0]  StiffnessAndInertiaType=CalculateFromGeometry  TopFlangeThickness=col_ft  TopFlangeThicknessUnits=m  TopFlangeWidth=col_fw  TopFlangeWidthUnits=m  TorsionalRigidity=1  TorsionalRigidityUnits=Pa*m^4  GraphicVisPropType=SimpleVisualProperties  WebThickness=col_wt  WebThicknessUnits=m  YoungsModulus=E_steel  YoungsModulusUnits=Pa  ProportionalDampingAlpha=0  ProportionalDampingAlphaUnits=1/s  ProportionalDampingBeta=0.001  ProportionalDampingBetaUnits=s  UniformModalDampingRatio=uni_dr
  ColumnRF1 : sm_lib/Body Elements/Flexible Bodies/Beams/Flexible I Beam  GraphicAmbientColor=[0.15 0.15 0.15 1.0]  AxialRigidity=1  AxialRigidityUnits=Pa*m^2  BendingCentroid=[0 0]  BendingCentroidUnits=m  FlexuralRigidity=[1 1]  FlexuralRigidityUnits=Pa*m^4  BottomFlangeThickness=col_ft  BottomFlangeThicknessUnits=m  BottomFlangeWidth=col_fw  BottomFlangeWidthUnits=m  CenterOfMass=[0 0]  CenterOfMassUnits=m  GraphicDiffuseColor=[0.5 0.5 0.5]  CrossFlexuralRigidity=0  CrossFlexuralRigidityUnits=Pa*m^4  SerializedFrames=<Frames><Frame><Id>Frame1</Id><Value><Name>Middle</Name><Origin><Source>ReferenceFrame</Source><FeatureName></FeatureName></Origin><PrimaryAxis><DefinedDirection>+Z</DefinedDirection><Source>ReferenceFrame</Source><SourceDirection>+Z</SourceDirection><FeatureName></FeatureName></PrimaryAxis><SecondaryAxis><DefinedDirection>+X</DefinedDirection><Source>ReferenceFrame</Source><SourceDirection>+X</SourceDirection><FeatureName></FeatureName></SecondaryAxis></Value></Frame></Frames>  DampingType=UniformModal  Density=rho_steel  DensityUnits=kg/m^3  DoExposeZmaxFrame=on  DoExposeZminFrame=on  GraphicEmissiveColor=[0.0 0.0 0.0 1.0]  GeometricCentroid=[0 0]  GeometricCentroidUnits=m  GraphicType=FromGeometry  EndToEndHeight=col_depth  EndToEndHeightUnits=m  Length=L_col  LengthUnits=m  MassMomentOfInertiaDensity=[1 1]  MassMomentOfInertiaDensityUnits=kg*m  MassPerUnitLength=1  MassPerUnitLengthUnits=kg/m  MassProductOfInertiaDensity=0  MassProductOfInertiaDensityUnits=kg*m  ModuliType=YoungsPoissons  NumElements=2  NumRetainedModes=1  GraphicOpacity=1.0  PoissonsRatio=p_steel  ReductionType=None  ShearCenter=[0 0]  ShearCenterUnits=m  ShearModulus=26  ShearModulusUnits=GPa  GraphicShininess=75  GraphicSpecularColor=[0.5 0.5 0.5 1.0]  StiffnessAndInertiaType=CalculateFromGeometry  TopFlangeThickness=col_ft  TopFlangeThicknessUnits=m  TopFlangeWidth=col_fw  TopFlangeWidthUnits=m  TorsionalRigidity=1  TorsionalRigidityUnits=Pa*m^4  GraphicVisPropType=SimpleVisualProperties  WebThickness=col_wt  WebThicknessUnits=m  YoungsModulus=E_steel  YoungsModulusUnits=Pa  ProportionalDampingAlpha=0  ProportionalDampingAlphaUnits=1/s  ProportionalDampingBeta=0.001  ProportionalDampingBetaUnits=s  UniformModalDampingRatio=uni_dr
  ColumnRF2 : sm_lib/Body Elements/Flexible Bodies/Beams/Flexible I Beam  GraphicAmbientColor=[0.15 0.15 0.15 1.0]  AxialRigidity=1  AxialRigidityUnits=Pa*m^2  BendingCentroid=[0 0]  BendingCentroidUnits=m  FlexuralRigidity=[1 1]  FlexuralRigidityUnits=Pa*m^4  BottomFlangeThickness=col_ft  BottomFlangeThicknessUnits=m  BottomFlangeWidth=col_fw  BottomFlangeWidthUnits=m  CenterOfMass=[0 0]  CenterOfMassUnits=m  GraphicDiffuseColor=[0.5 0.5 0.5]  CrossFlexuralRigidity=0  CrossFlexuralRigidityUnits=Pa*m^4  SerializedFrames=<Frames/>  DampingType=UniformModal  Density=rho_steel  DensityUnits=kg/m^3  DoExposeZmaxFrame=on  DoExposeZminFrame=on  GraphicEmissiveColor=[0.0 0.0 0.0 1.0]  GeometricCentroid=[0 0]  GeometricCentroidUnits=m  GraphicType=FromGeometry  EndToEndHeight=col_depth  EndToEndHeightUnits=m  Length=L_col2  LengthUnits=m  MassMomentOfInertiaDensity=[1 1]  MassMomentOfInertiaDensityUnits=kg*m  MassPerUnitLength=1  MassPerUnitLengthUnits=kg/m  MassProductOfInertiaDensity=0  MassProductOfInertiaDensityUnits=kg*m  ModuliType=YoungsPoissons  NumElements=1  NumRetainedModes=1  GraphicOpacity=1.0  PoissonsRatio=p_steel  ReductionType=None  ShearCenter=[0 0]  ShearCenterUnits=m  ShearModulus=26  ShearModulusUnits=GPa  GraphicShininess=75  GraphicSpecularColor=[0.5 0.5 0.5 1.0]  StiffnessAndInertiaType=CalculateFromGeometry  TopFlangeThickness=col_ft  TopFlangeThicknessUnits=m  TopFlangeWidth=col_fw  TopFlangeWidthUnits=m  TorsionalRigidity=1  TorsionalRigidityUnits=Pa*m^4  GraphicVisPropType=SimpleVisualProperties  WebThickness=col_wt  WebThicknessUnits=m  YoungsModulus=E_steel  YoungsModulusUnits=Pa  ProportionalDampingAlpha=0  ProportionalDampingAlphaUnits=1/s  ProportionalDampingBeta=0.001  ProportionalDampingBetaUnits=s  UniformModalDampingRatio=uni_dr
  ColumnRF3 : sm_lib/Body Elements/Flexible Bodies/Beams/Flexible I Beam  GraphicAmbientColor=[0.15 0.15 0.15 1.0]  AxialRigidity=1  AxialRigidityUnits=Pa*m^2  BendingCentroid=[0 0]  BendingCentroidUnits=m  FlexuralRigidity=[1 1]  FlexuralRigidityUnits=Pa*m^4  BottomFlangeThickness=col_ft  BottomFlangeThicknessUnits=m  BottomFlangeWidth=col_fw  BottomFlangeWidthUnits=m  CenterOfMass=[0 0]  CenterOfMassUnits=m  GraphicDiffuseColor=[0.5 0.5 0.5]  CrossFlexuralRigidity=0  CrossFlexuralRigidityUnits=Pa*m^4  SerializedFrames=<Frames/>  DampingType=UniformModal  Density=rho_steel  DensityUnits=kg/m^3  DoExposeZmaxFrame=on  DoExposeZminFrame=on  GraphicEmissiveColor=[0.0 0.0 0.0 1.0]  GeometricCentroid=[0 0]  GeometricCentroidUnits=m  GraphicType=FromGeometry  EndToEndHeight=col_depth  EndToEndHeightUnits=m  Length=L_col3  LengthUnits=m  MassMomentOfInertiaDensity=[1 1]  MassMomentOfInertiaDensityUnits=kg*m  MassPerUnitLength=1  MassPerUnitLengthUnits=kg/m  MassProductOfInertiaDensity=0  MassProductOfInertiaDensityUnits=kg*m  ModuliType=YoungsPoissons  NumElements=1  NumRetainedModes=1  GraphicOpacity=1.0  PoissonsRatio=p_steel  ReductionType=None  ShearCenter=[0 0]  ShearCenterUnits=m  ShearModulus=26  ShearModulusUnits=GPa  GraphicShininess=75  GraphicSpecularColor=[0.5 0.5 0.5 1.0]  StiffnessAndInertiaType=CalculateFromGeometry  TopFlangeThickness=col_ft  TopFlangeThicknessUnits=m  TopFlangeWidth=col_fw  TopFlangeWidthUnits=m  TorsionalRigidity=1  TorsionalRigidityUnits=Pa*m^4  GraphicVisPropType=SimpleVisualProperties  WebThickness=col_wt  WebThicknessUnits=m  YoungsModulus=E_steel  YoungsModulusUnits=Pa  ProportionalDampingAlpha=0  ProportionalDampingAlphaUnits=1/s  ProportionalDampingBeta=0.001  ProportionalDampingBetaUnits=s  UniformModalDampingRatio=uni_dr
  Constant{2,4..7,10} (6 alike) : Constant  Commented=on
  External Force and Torque2 : sm_lib/Forces and Torques/External Force and Torque  Commented=on  ForceResolutionFrame=AttachedFrame  EnableForceX=on  EnableForceY=on  EnableForceZ=on  EnableForce=off  TorqueResolutionFrame=AttachedFrame  EnableTorqueX=on  EnableTorqueY=on  EnableTorqueZ=on  EnableTorque=off
  File Log : slrealtimeloglib/File Log  Commented=on  decimation=50  inputProcessing=Elements as channels (sample based)
  File Log01 : slrealtimeloglib/File Log  Commented=on  decimation=50  inputProcessing=Elements as channels (sample based)
  File Log02 : slrealtimeloglib/File Log  Commented=on  decimation=50  inputProcessing=Elements as channels (sample based)
  File Log03 : slrealtimeloglib/File Log  Commented=on  decimation=50  inputProcessing=Elements as channels (sample based)
  Girder{1,3..16,18} (16 alike) : sm_lib/Body Elements/Flexible Bodies/Beams/Flexible I Beam  GraphicAmbientColor=[0.15 0.15 0.15 1.0]  AxialRigidity=1  AxialRigidityUnits=Pa*m^2  BendingCentroid=[0 0]  BendingCentroidUnits=m  FlexuralRigidity=[1 1]  FlexuralRigidityUnits=Pa*m^4  BottomFlangeThickness=beam_ft  BottomFlangeThicknessUnits=m  BottomFlangeWidth=beam_fw  BottomFlangeWidthUnits=m  CenterOfMass=[0 0]  CenterOfMassUnits=m  GraphicDiffuseColor=[0.5 0.5 0.5]  CrossFlexuralRigidity=0  CrossFlexuralRigidityUnits=Pa*m^4  SerializedFrames=<Frames/>  DampingType=UniformModal  Density=rho_steel  DensityUnits=kg/m^3  DoExposeZmaxFrame=on  DoExposeZminFrame=on  GraphicEmissiveColor=[0.0 0.0 0.0 1.0]  GeometricCentroid=[0 0]  GeometricCentroidUnits=m  GraphicType=FromGeometry  EndToEndHeight=beam_depth  EndToEndHeightUnits=m  Length=L_beam  LengthUnits=m  MassMomentOfInertiaDensity=[1 1]  MassMomentOfInertiaDensityUnits=kg*m  MassPerUnitLength=1  MassPerUnitLengthUnits=kg/m  MassProductOfInertiaDensity=0  MassProductOfInertiaDensityUnits=kg*m  ModuliType=YoungsPoissons  NumElements=1  NumRetainedModes=1  GraphicOpacity=1.0  PoissonsRatio=p_steel  ReductionType=None  ShearCenter=[0 0]  ShearCenterUnits=m  ShearModulus=26  ShearModulusUnits=GPa  GraphicShininess=75  GraphicSpecularColor=[0.5 0.5 0.5 1.0]  StiffnessAndInertiaType=CalculateFromGeometry  TopFlangeThickness=beam_ft  TopFlangeThicknessUnits=m  TopFlangeWidth=beam_fw  TopFlangeWidthUnits=m  TorsionalRigidity=1  TorsionalRigidityUnits=Pa*m^4  GraphicVisPropType=SimpleVisualProperties  WebThickness=beam_wt  WebThicknessUnits=m  YoungsModulus=E_steel  YoungsModulusUnits=Pa  ProportionalDampingAlpha=0  ProportionalDampingAlphaUnits=1/s  ProportionalDampingBeta=0.001  ProportionalDampingBetaUnits=s  UniformModalDampingRatio=uni_dr
  Girder17 : sm_lib/Body Elements/Flexible Bodies/Beams/Flexible I Beam  GraphicAmbientColor=[0.15 0.15 0.15 1.0]  AxialRigidity=1  AxialRigidityUnits=Pa*m^2  BendingCentroid=[0 0]  BendingCentroidUnits=m  FlexuralRigidity=[1 1]  FlexuralRigidityUnits=Pa*m^4  BottomFlangeThickness=beam_ft  BottomFlangeThicknessUnits=m  BottomFlangeWidth=beam_fw  BottomFlangeWidthUnits=m  CenterOfMass=[0 0]  CenterOfMassUnits=m  GraphicDiffuseColor=[0.5 0.5 0.5]  CrossFlexuralRigidity=0  CrossFlexuralRigidityUnits=Pa*m^4  SerializedFrames=<Frames><Frame><Id>Frame1</Id><Value><Name>Middle</Name><Origin><Source>ReferenceFrame</Source><FeatureName></FeatureName></Origin><PrimaryAxis><DefinedDirection>+Z</DefinedDirection><Source>ReferenceFrame</Source><SourceDirection>+Z</SourceDirection><FeatureName></FeatureName></PrimaryAxis><SecondaryAxis><DefinedDirection>+X</DefinedDirection><Source>ReferenceFrame</Source><SourceDirection>+X</SourceDirection><FeatureName></FeatureName></SecondaryAxis></Value></Frame></Frames>  DampingType=UniformModal  Density=rho_steel  DensityUnits=kg/m^3  DoExposeZmaxFrame=on  DoExposeZminFrame=on  GraphicEmissiveColor=[0.0 0.0 0.0 1.0]  GeometricCentroid=[0 0]  GeometricCentroidUnits=m  GraphicType=FromGeometry  EndToEndHeight=beam_depth  EndToEndHeightUnits=m  Length=L_beam  LengthUnits=m  MassMomentOfInertiaDensity=[1 1]  MassMomentOfInertiaDensityUnits=kg*m  MassPerUnitLength=1  MassPerUnitLengthUnits=kg/m  MassProductOfInertiaDensity=0  MassProductOfInertiaDensityUnits=kg*m  ModuliType=YoungsPoissons  NumElements=2  NumRetainedModes=1  GraphicOpacity=1.0  PoissonsRatio=p_steel  ReductionType=None  ShearCenter=[0 0]  ShearCenterUnits=m  ShearModulus=26  ShearModulusUnits=GPa  GraphicShininess=75  GraphicSpecularColor=[0.5 0.5 0.5 1.0]  StiffnessAndInertiaType=CalculateFromGeometry  TopFlangeThickness=beam_ft  TopFlangeThicknessUnits=m  TopFlangeWidth=beam_fw  TopFlangeWidthUnits=m  TorsionalRigidity=1  TorsionalRigidityUnits=Pa*m^4  GraphicVisPropType=SimpleVisualProperties  WebThickness=beam_wt  WebThicknessUnits=m  YoungsModulus=E_steel  YoungsModulusUnits=Pa  ProportionalDampingAlpha=0  ProportionalDampingAlphaUnits=1/s  ProportionalDampingBeta=0.001  ProportionalDampingBetaUnits=s  UniformModalDampingRatio=uni_dr
  Girder2 : sm_lib/Body Elements/Flexible Bodies/Beams/Flexible I Beam  GraphicAmbientColor=[0.15 0.15 0.15 1.0]  AxialRigidity=1  AxialRigidityUnits=Pa*m^2  BendingCentroid=[0 0]  BendingCentroidUnits=m  FlexuralRigidity=[1 1]  FlexuralRigidityUnits=Pa*m^4  BottomFlangeThickness=beam_ft  BottomFlangeThicknessUnits=m  BottomFlangeWidth=beam_fw  BottomFlangeWidthUnits=m  CenterOfMass=[0 0]  CenterOfMassUnits=m  GraphicDiffuseColor=[0.5 0.5 0.5]  CrossFlexuralRigidity=0  CrossFlexuralRigidityUnits=Pa*m^4  SerializedFrames=<Frames><Frame><Id>Frame1</Id><Value><Name>Middle</Name><Origin><Source>ReferenceFrame</Source><FeatureName></FeatureName></Origin><PrimaryAxis><DefinedDirection>+Z</DefinedDirection><Source>ReferenceFrame</Source><SourceDirection>+Z</SourceDirection><FeatureName></FeatureName></PrimaryAxis><SecondaryAxis><DefinedDirection>+X</DefinedDirection><Source>ReferenceFrame</Source><SourceDirection>+X</SourceDirection><FeatureName></FeatureName></SecondaryAxis></Value></Frame></Frames>  DampingType=UniformModal  Density=rho_steel  DensityUnits=kg/m^3  DoExposeZmaxFrame=on  DoExposeZminFrame=on  GraphicEmissiveColor=[0.0 0.0 0.0 1.0]  GeometricCentroid=[0 0]  GeometricCentroidUnits=m  GraphicType=FromGeometry  EndToEndHeight=beam_depth  EndToEndHeightUnits=m  Length=L_beam  LengthUnits=m  MassMomentOfInertiaDensity=[1 1]  MassMomentOfInertiaDensityUnits=kg*m  MassPerUnitLength=1  MassPerUnitLengthUnits=kg/m  MassProductOfInertiaDensity=0  MassProductOfInertiaDensityUnits=kg*m  ModuliType=YoungsPoissons  NumElements=2  NumRetainedModes=1  GraphicOpacity=1.0  PoissonsRatio=p_steel  ReductionType=None  ShearCenter=[0 0]  ShearCenterUnits=m  ShearModulus=26  ShearModulusUnits=GPa  GraphicShininess=75  GraphicSpecularColor=[0.5 0.5 0.5 1.0]  StiffnessAndInertiaType=CalculateFromGeometry  TopFlangeThickness=beam_ft  TopFlangeThicknessUnits=m  TopFlangeWidth=beam_fw  TopFlangeWidthUnits=m  TorsionalRigidity=1  TorsionalRigidityUnits=Pa*m^4  GraphicVisPropType=SimpleVisualProperties  WebThickness=beam_wt  WebThicknessUnits=m  YoungsModulus=E_steel  YoungsModulusUnits=Pa  ProportionalDampingAlpha=0  ProportionalDampingAlphaUnits=1/s  ProportionalDampingBeta=0.001  ProportionalDampingBetaUnits=s  UniformModalDampingRatio=uni_dr
  K bracing{,1..3} (4 alike) : sm_lib/Body Elements/Flexible Bodies/Beams/Flexible I Beam  GraphicAmbientColor=[0.15 0.15 0.15 1.0]  AxialRigidity=1  AxialRigidityUnits=Pa*m^2  BendingCentroid=[0 0]  BendingCentroidUnits=m  FlexuralRigidity=[1 1]  FlexuralRigidityUnits=Pa*m^4  BottomFlangeThickness=beam_ft  BottomFlangeThicknessUnits=m  BottomFlangeWidth=beam_fw  BottomFlangeWidthUnits=m  CenterOfMass=[0 0]  CenterOfMassUnits=m  GraphicDiffuseColor=[0.5 0.5 0.5]  CrossFlexuralRigidity=0  CrossFlexuralRigidityUnits=Pa*m^4  SerializedFrames=<Frames/>  DampingType=UniformModal  Density=rho_steel  DensityUnits=kg/m^3  DoExposeZmaxFrame=on  DoExposeZminFrame=on  GraphicEmissiveColor=[0.0 0.0 0.0 1.0]  GeometricCentroid=[0 0]  GeometricCentroidUnits=m  GraphicType=FromGeometry  EndToEndHeight=beam_depth  EndToEndHeightUnits=m  Length=L_brace  LengthUnits=m  MassMomentOfInertiaDensity=[1 1]  MassMomentOfInertiaDensityUnits=kg*m  MassPerUnitLength=1  MassPerUnitLengthUnits=kg/m  MassProductOfInertiaDensity=0  MassProductOfInertiaDensityUnits=kg*m  ModuliType=YoungsPoissons  NumElements=1  NumRetainedModes=1  GraphicOpacity=1.0  PoissonsRatio=p_steel  ReductionType=None  ShearCenter=[0 0]  ShearCenterUnits=m  ShearModulus=26  ShearModulusUnits=GPa  GraphicShininess=75  GraphicSpecularColor=[0.5 0.5 0.5 1.0]  StiffnessAndInertiaType=CalculateFromGeometry  TopFlangeThickness=beam_ft  TopFlangeThicknessUnits=m  TopFlangeWidth=beam_fw  TopFlangeWidthUnits=m  TorsionalRigidity=1  TorsionalRigidityUnits=Pa*m^4  GraphicVisPropType=SimpleVisualProperties  WebThickness=beam_wt  WebThicknessUnits=m  YoungsModulus=E_steel  YoungsModulusUnits=Pa  ProportionalDampingAlpha=0  ProportionalDampingAlphaUnits=1/s  ProportionalDampingBeta=0.001  ProportionalDampingBetaUnits=s  UniformModalDampingRatio=uni_dr
  LFColDepPosition : slrealtimeloglib/File Log  decimation=200  inputProcessing=Elements as channels (sample based)
  LFColHorPosition : slrealtimeloglib/File Log  decimation=200  inputProcessing=Elements as channels (sample based)
  LFColMove : sm_lib/Frames and Transforms/Transform Sensor  MeasurementFrame=Base  RotationSequence=XYX  SenseAngle=off  SenseAxis=off  SenseQ=off  SenseR=off  SenseRotationSequence=off  SenseOmegaX=off  SenseOmegaY=off  SenseOmegaZ=off  SenseQDot=off  SenseRDot=off  SenseRotationSequenceDot=off  SenseAlphaX=off  SenseAlphaY=off  SenseAlphaZ=off  SenseQDDot=off  SenseRDDot=off  SenseX=on  SenseY=on  SenseZ=on  SenseRad=off  SenseAzim=off  SenseDist=off  SenseInc=off  SenseXDot=off  SenseYDot=off  SenseZDot=off  SenseRadDot=off  SenseAzimDot=off  SenseDistDot=off  SenseIncDot=off  SenseXDDot=off  SenseYDDot=off  SenseZDDot=off  SenseRadDDot=off  SenseAzimDDot=off  SenseDistDDot=off  SenseIncDDot=off
  LFColVertiPosition : slrealtimeloglib/File Log  decimation=200  inputProcessing=Elements as channels (sample based)
  PS-Simulink Converter{1,5..6,19} (4 alike) : nesl_utility/PS-Simulink Converter  Commented=on  PhysicalDomain=network_engine_domain  SubClassName=ps_output  LeftPortType=input  RightPortType=output  PseudoPeriodic=off  Frequencies=[]  VectorFormat=1-D array  Unit=inherit  AffineConversion=off
  PS-Simulink Converter{2..4,7..12} (9 alike) : nesl_utility/PS-Simulink Converter  PhysicalDomain=network_engine_domain  SubClassName=ps_output  LeftPortType=input  RightPortType=output  PseudoPeriodic=off  Frequencies=[]  VectorFormat=1-D array  Unit=inherit  AffineConversion=off
  Quaternions to Rotation Angles1 : sharedtransform/Quaternions to Rotation Angles  Commented=on  rotationOrder=XYZ  aMode=aMode
  RFColDepPosition : slrealtimeloglib/File Log  decimation=200  inputProcessing=Elements as channels (sample based)
  RFColHorPosition : slrealtimeloglib/File Log  decimation=200  inputProcessing=Elements as channels (sample based)
  RFColMove : sm_lib/Frames and Transforms/Transform Sensor  MeasurementFrame=Base  RotationSequence=XYX  SenseAngle=off  SenseAxis=off  SenseQ=off  SenseR=off  SenseRotationSequence=off  SenseOmegaX=off  SenseOmegaY=off  SenseOmegaZ=off  SenseQDot=off  SenseRDot=off  SenseRotationSequenceDot=off  SenseAlphaX=off  SenseAlphaY=off  SenseAlphaZ=off  SenseQDDot=off  SenseRDDot=off  SenseX=on  SenseY=on  SenseZ=on  SenseRad=off  SenseAzim=off  SenseDist=off  SenseInc=off  SenseXDot=off  SenseYDot=off  SenseZDot=off  SenseRadDot=off  SenseAzimDot=off  SenseDistDot=off  SenseIncDot=off  SenseXDDot=off  SenseYDDot=off  SenseZDDot=off  SenseRadDDot=off  SenseAzimDDot=off  SenseDistDDot=off  SenseIncDDot=off
  RFColVertiPosition : slrealtimeloglib/File Log  decimation=200  inputProcessing=Elements as channels (sample based)
  Rigid Transform{,1,3,5..7,10..15} (12 alike) : sm_lib/Frames and Transforms/Rigid Transform  TranslationMethod=None  TranslationStandardOffset=0  TranslationStandardOffsetUnits=m  TranslationStandardAxis=+Z  TranslationCartesianOffset=[0 0 0]  TranslationCartesianOffsetUnits=m  TranslationROffset=0  TranslationROffsetUnits=m  TranslationZOffset=0  TranslationZOffsetUnits=m  TranslationThetaOffset=0  TranslationThetaOffsetUnits=deg  RotationMethod=AlignedAxes  RotationAngleUnits=deg  RotationStandardAxis=+Z  RotationAngle=0.0  RotationArbitraryAxis=[0 0 1]  FollAlignAxisA=+Y  BaseAlignAxisA=+Z  FollAlignAxisB=+Z  BaseAlignAxisB=+X  RotationSequenceAxes=FollowerAxes  RotationSequence=XYX  RotationSequenceAngles=[0 0 0]  RotationSequenceAnglesUnits=deg  RotationMatrix=[1 0 0; 0 1 0; 0 0 1]  Quaternion=[1 0 0 0]
  Rigid Transform{16..27} (12 alike) : sm_lib/Frames and Transforms/Rigid Transform  TranslationMethod=None  TranslationStandardOffset=0  TranslationStandardOffsetUnits=m  TranslationStandardAxis=+Z  TranslationCartesianOffset=[0 0 0]  TranslationCartesianOffsetUnits=m  TranslationROffset=0  TranslationROffsetUnits=m  TranslationZOffset=0  TranslationZOffsetUnits=m  TranslationThetaOffset=0  TranslationThetaOffsetUnits=deg  RotationMethod=AlignedAxes  RotationAngleUnits=deg  RotationStandardAxis=+Z  RotationAngle=0.0  RotationArbitraryAxis=[0 0 1]  FollAlignAxisA=+Y  BaseAlignAxisA=+Z  FollAlignAxisB=+Z  BaseAlignAxisB=+Y  RotationSequenceAxes=FollowerAxes  RotationSequence=XYX  RotationSequenceAngles=[0 0 0]  RotationSequenceAnglesUnits=deg  RotationMatrix=[1 0 0; 0 1 0; 0 0 1]  Quaternion=[1 0 0 0]
  Rigid Transform{2,4,8..9,29,31,33,35,37..38,41,43..44,47,49,51} (16 alike) : sm_lib/Frames and Transforms/Rigid Transform  TranslationMethod=None  TranslationStandardOffset=0  TranslationStandardOffsetUnits=m  TranslationStandardAxis=+Z  TranslationCartesianOffset=[0 0 0]  TranslationCartesianOffsetUnits=m  TranslationROffset=0  TranslationROffsetUnits=m  TranslationZOffset=0  TranslationZOffsetUnits=m  TranslationThetaOffset=0  TranslationThetaOffsetUnits=deg  RotationMethod=AlignedAxes  RotationAngleUnits=deg  RotationStandardAxis=+Z  RotationAngle=0.0  RotationArbitraryAxis=[0 0 1]  FollAlignAxisA=+Z  BaseAlignAxisA=+Z  FollAlignAxisB=+Y  BaseAlignAxisB=+X  RotationSequenceAxes=FollowerAxes  RotationSequence=XYX  RotationSequenceAngles=[0 0 0]  RotationSequenceAnglesUnits=deg  RotationMatrix=[1 0 0; 0 1 0; 0 0 1]  Quaternion=[1 0 0 0]
  Rigid Transform{28,30,32,34,36,39..40,42,45..46,48,50} (12 alike) : sm_lib/Frames and Transforms/Rigid Transform  TranslationMethod=None  TranslationStandardOffset=0  TranslationStandardOffsetUnits=m  TranslationStandardAxis=+Z  TranslationCartesianOffset=[0 0 0]  TranslationCartesianOffsetUnits=m  TranslationROffset=0  TranslationROffsetUnits=m  TranslationZOffset=0  TranslationZOffsetUnits=m  TranslationThetaOffset=0  TranslationThetaOffsetUnits=deg  RotationMethod=AlignedAxes  RotationAngleUnits=deg  RotationStandardAxis=+Z  RotationAngle=0.0  RotationArbitraryAxis=[0 0 1]  FollAlignAxisA=+Z  BaseAlignAxisA=+Y  FollAlignAxisB=+Y  BaseAlignAxisB=+Z  RotationSequenceAxes=FollowerAxes  RotationSequence=XYX  RotationSequenceAngles=[0 0 0]  RotationSequenceAnglesUnits=deg  RotationMatrix=[1 0 0; 0 1 0; 0 0 1]  Quaternion=[1 0 0 0]
  Rigid Transform52 : sm_lib/Frames and Transforms/Rigid Transform  TranslationMethod=None  TranslationStandardOffset=0  TranslationStandardOffsetUnits=m  TranslationStandardAxis=+Z  TranslationCartesianOffset=[0.3 0 0]  TranslationCartesianOffsetUnits=m  TranslationROffset=0  TranslationROffsetUnits=m  TranslationZOffset=0  TranslationZOffsetUnits=m  TranslationThetaOffset=0  TranslationThetaOffsetUnits=deg  RotationMethod=StandardAxis  RotationAngleUnits=rad  RotationStandardAxis=+X  RotationAngle=frame_rot+pi  RotationArbitraryAxis=[0 0 1]  FollAlignAxisA=+Y  BaseAlignAxisA=+Z  FollAlignAxisB=+Z  BaseAlignAxisB=+X  RotationSequenceAxes=FollowerAxes  RotationSequence=XYX  RotationSequenceAngles=[0 0 0]  RotationSequenceAnglesUnits=deg  RotationMatrix=[1 0 0; 0 1 0; 0 0 1]  Quaternion=[1 0 0 0]
  Rigid Transform{53,58,61,64} (4 alike) : sm_lib/Frames and Transforms/Rigid Transform  TranslationMethod=None  TranslationStandardOffset=0  TranslationStandardOffsetUnits=m  TranslationStandardAxis=+Z  TranslationCartesianOffset=[0.3 0 0]  TranslationCartesianOffsetUnits=m  TranslationROffset=0  TranslationROffsetUnits=m  TranslationZOffset=0  TranslationZOffsetUnits=m  TranslationThetaOffset=0  TranslationThetaOffsetUnits=deg  RotationMethod=AlignedAxes  RotationAngleUnits=rad  RotationStandardAxis=+X  RotationAngle=frame_rot+pi  RotationArbitraryAxis=[0 0 1]  FollAlignAxisA=-X  BaseAlignAxisA=+X  FollAlignAxisB=-Y  BaseAlignAxisB=+Y  RotationSequenceAxes=FollowerAxes  RotationSequence=XYX  RotationSequenceAngles=[0 0 0]  RotationSequenceAnglesUnits=deg  RotationMatrix=[1 0 0; 0 1 0; 0 0 1]  Quaternion=[1 0 0 0]
  Rigid Transform54 : sm_lib/Frames and Transforms/Rigid Transform  TranslationMethod=None  TranslationStandardOffset=0  TranslationStandardOffsetUnits=m  TranslationStandardAxis=+Z  TranslationCartesianOffset=[0 0.2 0.2]  TranslationCartesianOffsetUnits=m  TranslationROffset=0  TranslationROffsetUnits=m  TranslationZOffset=0  TranslationZOffsetUnits=m  TranslationThetaOffset=0  TranslationThetaOffsetUnits=deg  RotationMethod=StandardAxis  RotationAngleUnits=rad  RotationStandardAxis=+X  RotationAngle=pi/2-frame_rot  RotationArbitraryAxis=[0 0 1]  FollAlignAxisA=+X  BaseAlignAxisA=+Y  FollAlignAxisB=+Y  BaseAlignAxisB=+Z  RotationSequenceAxes=FollowerAxes  RotationSequence=XYX  RotationSequenceAngles=[0 0 0]  RotationSequenceAnglesUnits=deg  RotationMatrix=[1 0 0; 0 1 0; 0 0 1]  Quaternion=[1 0 0 0]
  Rigid Transform55 : sm_lib/Frames and Transforms/Rigid Transform  Commented=on  TranslationMethod=None  TranslationStandardOffset=0  TranslationStandardOffsetUnits=m  TranslationStandardAxis=+Z  TranslationCartesianOffset=[0 0 0]  TranslationCartesianOffsetUnits=m  TranslationROffset=0  TranslationROffsetUnits=m  TranslationZOffset=0  TranslationZOffsetUnits=m  TranslationThetaOffset=0  TranslationThetaOffsetUnits=deg  RotationMethod=StandardAxis  RotationAngleUnits=rad  RotationStandardAxis=+X  RotationAngle=pi/2-frame_rot  RotationArbitraryAxis=[0 0 1]  FollAlignAxisA=+Y  BaseAlignAxisA=+Z  FollAlignAxisB=+Z  BaseAlignAxisB=+X  RotationSequenceAxes=FollowerAxes  RotationSequence=XYX  RotationSequenceAngles=[0 0 0]  RotationSequenceAnglesUnits=deg  RotationMatrix=[1 0 0; 0 1 0; 0 0 1]  Quaternion=[1 0 0 0]
  Rigid Transform56 : sm_lib/Frames and Transforms/Rigid Transform  Commented=on  TranslationMethod=None  TranslationStandardOffset=0  TranslationStandardOffsetUnits=m  TranslationStandardAxis=+Z  TranslationCartesianOffset=[0 0 0]  TranslationCartesianOffsetUnits=m  TranslationROffset=0  TranslationROffsetUnits=m  TranslationZOffset=0  TranslationZOffsetUnits=m  TranslationThetaOffset=0  TranslationThetaOffsetUnits=deg  RotationMethod=AlignedAxes  RotationAngleUnits=rad  RotationStandardAxis=+X  RotationAngle=pi/2-frame_rot  RotationArbitraryAxis=[0 0 1]  FollAlignAxisA=-X  BaseAlignAxisA=+X  FollAlignAxisB=+Y  BaseAlignAxisB=+Y  RotationSequenceAxes=FollowerAxes  RotationSequence=XYX  RotationSequenceAngles=[0 0 0]  RotationSequenceAnglesUnits=deg  RotationMatrix=[1 0 0; 0 1 0; 0 0 1]  Quaternion=[1 0 0 0]
  Rigid Transform57 : sm_lib/Frames and Transforms/Rigid Transform  TranslationMethod=None  TranslationStandardOffset=0  TranslationStandardOffsetUnits=m  TranslationStandardAxis=+Z  TranslationCartesianOffset=[0.3 0 0]  TranslationCartesianOffsetUnits=m  TranslationROffset=0  TranslationROffsetUnits=m  TranslationZOffset=0  TranslationZOffsetUnits=m  TranslationThetaOffset=0  TranslationThetaOffsetUnits=deg  RotationMethod=StandardAxis  RotationAngleUnits=rad  RotationStandardAxis=-X  RotationAngle=frame_rot  RotationArbitraryAxis=[0 0 1]  FollAlignAxisA=+Y  BaseAlignAxisA=+Z  FollAlignAxisB=+Z  BaseAlignAxisB=+X  RotationSequenceAxes=FollowerAxes  RotationSequence=XYX  RotationSequenceAngles=[0 0 0]  RotationSequenceAnglesUnits=deg  RotationMatrix=[1 0 0; 0 1 0; 0 0 1]  Quaternion=[1 0 0 0]
  Rigid Transform59 : sm_lib/Frames and Transforms/Rigid Transform  TranslationMethod=None  TranslationStandardOffset=0  TranslationStandardOffsetUnits=m  TranslationStandardAxis=+Z  TranslationCartesianOffset=[0 0.2 0.2]  TranslationCartesianOffsetUnits=m  TranslationROffset=0  TranslationROffsetUnits=m  TranslationZOffset=0  TranslationZOffsetUnits=m  TranslationThetaOffset=0  TranslationThetaOffsetUnits=deg  RotationMethod=StandardAxis  RotationAngleUnits=rad  RotationStandardAxis=-X  RotationAngle=pi/2-frame_rot  RotationArbitraryAxis=[0 0 1]  FollAlignAxisA=+X  BaseAlignAxisA=+Y  FollAlignAxisB=+Y  BaseAlignAxisB=+Z  RotationSequenceAxes=FollowerAxes  RotationSequence=XYX  RotationSequenceAngles=[0 0 0]  RotationSequenceAnglesUnits=deg  RotationMatrix=[1 0 0; 0 1 0; 0 0 1]  Quaternion=[1 0 0 0]
  Rigid Transform60 : sm_lib/Frames and Transforms/Rigid Transform  TranslationMethod=None  TranslationStandardOffset=0  TranslationStandardOffsetUnits=m  TranslationStandardAxis=+Z  TranslationCartesianOffset=[0.3 0 0]  TranslationCartesianOffsetUnits=m  TranslationROffset=0  TranslationROffsetUnits=m  TranslationZOffset=0  TranslationZOffsetUnits=m  TranslationThetaOffset=0  TranslationThetaOffsetUnits=deg  RotationMethod=StandardAxis  RotationAngleUnits=rad  RotationStandardAxis=+X  RotationAngle=frame_rot+pi  RotationArbitraryAxis=[0 0 1]  FollAlignAxisA=+Y  BaseAlignAxisA=+Z  FollAlignAxisB=+Z  BaseAlignAxisB=+X  RotationSequenceAxes=FollowerAxes  RotationSequence=XYX  RotationSequenceAngles=[0 0 0]  RotationSequenceAnglesUnits=deg  RotationMatrix=[1 0 0; 0 1 0; 0 0 1]  Quaternion=[1 0 0 0]
  Rigid Transform62 : sm_lib/Frames and Transforms/Rigid Transform  TranslationMethod=None  TranslationStandardOffset=0  TranslationStandardOffsetUnits=m  TranslationStandardAxis=+Z  TranslationCartesianOffset=[0 0.2 0.2]  TranslationCartesianOffsetUnits=m  TranslationROffset=0  TranslationROffsetUnits=m  TranslationZOffset=0  TranslationZOffsetUnits=m  TranslationThetaOffset=0  TranslationThetaOffsetUnits=deg  RotationMethod=StandardAxis  RotationAngleUnits=rad  RotationStandardAxis=+X  RotationAngle=pi/2-frame_rot  RotationArbitraryAxis=[0 0 1]  FollAlignAxisA=+X  BaseAlignAxisA=+Y  FollAlignAxisB=+Y  BaseAlignAxisB=+Z  RotationSequenceAxes=FollowerAxes  RotationSequence=XYX  RotationSequenceAngles=[0 0 0]  RotationSequenceAnglesUnits=deg  RotationMatrix=[1 0 0; 0 1 0; 0 0 1]  Quaternion=[1 0 0 0]
  Rigid Transform63 : sm_lib/Frames and Transforms/Rigid Transform  TranslationMethod=None  TranslationStandardOffset=0  TranslationStandardOffsetUnits=m  TranslationStandardAxis=+Z  TranslationCartesianOffset=[0.3 0 0]  TranslationCartesianOffsetUnits=m  TranslationROffset=0  TranslationROffsetUnits=m  TranslationZOffset=0  TranslationZOffsetUnits=m  TranslationThetaOffset=0  TranslationThetaOffsetUnits=deg  RotationMethod=StandardAxis  RotationAngleUnits=rad  RotationStandardAxis=-X  RotationAngle=frame_rot  RotationArbitraryAxis=[0 0 1]  FollAlignAxisA=+Y  BaseAlignAxisA=+Z  FollAlignAxisB=+Z  BaseAlignAxisB=+X  RotationSequenceAxes=FollowerAxes  RotationSequence=XYX  RotationSequenceAngles=[0 0 0]  RotationSequenceAnglesUnits=deg  RotationMatrix=[1 0 0; 0 1 0; 0 0 1]  Quaternion=[1 0 0 0]
  Rigid Transform65 : sm_lib/Frames and Transforms/Rigid Transform  TranslationMethod=None  TranslationStandardOffset=0  TranslationStandardOffsetUnits=m  TranslationStandardAxis=+Z  TranslationCartesianOffset=[0 0.2 0.2]  TranslationCartesianOffsetUnits=m  TranslationROffset=0  TranslationROffsetUnits=m  TranslationZOffset=0  TranslationZOffsetUnits=m  TranslationThetaOffset=0  TranslationThetaOffsetUnits=deg  RotationMethod=StandardAxis  RotationAngleUnits=rad  RotationStandardAxis=-X  RotationAngle=pi/2-frame_rot  RotationArbitraryAxis=[0 0 1]  FollAlignAxisA=+X  BaseAlignAxisA=+Y  FollAlignAxisB=+Y  BaseAlignAxisB=+Z  RotationSequenceAxes=FollowerAxes  RotationSequence=XYX  RotationSequenceAngles=[0 0 0]  RotationSequenceAnglesUnits=deg  RotationMatrix=[1 0 0; 0 1 0; 0 0 1]  Quaternion=[1 0 0 0]
  Rigid Transform{66,68,70,72,74,77} (6 alike) : sm_lib/Frames and Transforms/Rigid Transform  Commented=on  TranslationMethod=Cartesian  TranslationStandardOffset=0  TranslationStandardOffsetUnits=m  TranslationStandardAxis=+Z  TranslationCartesianOffset=[0 0 3*L_beam]  TranslationCartesianOffsetUnits=m  TranslationROffset=0  TranslationROffsetUnits=m  TranslationZOffset=0  TranslationZOffsetUnits=m  TranslationThetaOffset=0  TranslationThetaOffsetUnits=deg  RotationMethod=AlignedAxes  RotationAngleUnits=deg  RotationStandardAxis=+Z  RotationAngle=0.0  RotationArbitraryAxis=[0 0 1]  FollAlignAxisA=+X  BaseAlignAxisA=+X  FollAlignAxisB=+Z  BaseAlignAxisB=+Y  RotationSequenceAxes=FollowerAxes  RotationSequence=XYX  RotationSequenceAngles=[0 0 0]  RotationSequenceAnglesUnits=deg  RotationMatrix=[1 0 0; 0 1 0; 0 0 1]  Quaternion=[1 0 0 0]
  Rigid Transform{67,69,71,73,75..76} (6 alike) : sm_lib/Frames and Transforms/Rigid Transform  Commented=on  TranslationMethod=None  TranslationStandardOffset=0  TranslationStandardOffsetUnits=m  TranslationStandardAxis=+Z  TranslationCartesianOffset=[0 0 3*L_beam]  TranslationCartesianOffsetUnits=m  TranslationROffset=0  TranslationROffsetUnits=m  TranslationZOffset=0  TranslationZOffsetUnits=m  TranslationThetaOffset=0  TranslationThetaOffsetUnits=deg  RotationMethod=AlignedAxes  RotationAngleUnits=deg  RotationStandardAxis=+Z  RotationAngle=0.0  RotationArbitraryAxis=[0 0 1]  FollAlignAxisA=+X  BaseAlignAxisA=+X  FollAlignAxisB=+Z  BaseAlignAxisB=+Y  RotationSequenceAxes=FollowerAxes  RotationSequence=XYX  RotationSequenceAngles=[0 0 0]  RotationSequenceAnglesUnits=deg  RotationMatrix=[1 0 0; 0 1 0; 0 0 1]  Quaternion=[1 0 0 0]
  Simulink-PS Converter{2,4..7,10} (6 alike) : nesl_utility/Simulink-PS Converter  Commented=on  PhysicalDomain=network_engine_domain  SubClassName=ps_input  LeftPortType=input  RightPortType=output  PseudoPeriodic=off  Frequencies=[]  NoiseDistribution=none  NoiseParameters=[]  Unit=1  AffineConversion=off  FilteringAndDerivatives=provide  SimscapeFilterOrder=1  InputFilterTimeConstant=0.001  UdotUserProvided=0
  Weld Joint{,1..27} (28 alike) : sm_lib/Joints/Weld Joint  JointMode=Normal  SenseConstraintForce=off  SenseConstraintForceX=off  SenseConstraintForceY=off  SenseConstraintForceZ=off  SenseConstraintTorque=off  SenseConstraintTorqueX=off  SenseConstraintTorqueY=off  SenseConstraintTorqueZ=off  SenseTotalForce=off  SenseTotalForceX=off  SenseTotalForceY=off  SenseTotalForceZ=off  SenseTotalTorque=off  SenseTotalTorqueX=off  SenseTotalTorqueY=off  SenseTotalTorqueZ=off  CompositeWrenchDir=FollowerOnBase  CompositeWrenchFrame=BaseFrame
  LB : PMIOPort  Side=Left
  RB : PMIOPort  Port=2  Side=Left
  RF : PMIOPort  Port=3  Side=Left
  LF : PMIOPort  Port=4  Side=Left
  GroundSurface : PMIOPort  Port=5  Side=Left
  wires:
  Constant2/1 -> Simulink-PS Converter2/1
  Constant10/1 -> Simulink-PS Converter10/1
  Constant7/1 -> Simulink-PS Converter7/1
  Constant6/1 -> Simulink-PS Converter6/1
  Constant5/1 -> Simulink-PS Converter5/1
  Constant4/1 -> Simulink-PS Converter4/1
  PS-Simulink Converter19/1 -> File Log03/1
  PS-Simulink Converter6/1 -> Quaternions to Rotation Angles1/1
  PS-Simulink Converter5/1 -> File Log01/1
  PS-Simulink Converter1/1 -> File Log02/1
  Quaternions to Rotation Angles1/1 -> File Log/1
  PS-Simulink Converter2/1 -> RFColHorPosition/1
  PS-Simulink Converter3/1 -> RFColDepPosition/1
  PS-Simulink Converter4/1 -> RFColVertiPosition/1
  PS-Simulink Converter9/1 -> LFColVertiPosition/1
  PS-Simulink Converter8/1 -> LFColDepPosition/1
  PS-Simulink Converter7/1 -> LFColHorPosition/1
  PS-Simulink Converter12/1 -> 3rdFloorVertiPosition/1
  PS-Simulink Converter11/1 -> 3rdFloorDepPosition/1
  PS-Simulink Converter10/1 -> 3rdFloorHorPosition/1
  connections:
  ColumnRB2/LConn1 -- Weld Joint/RConn1
  ColumnRB3/LConn1 -- Weld Joint7/RConn1 -- Rigid Transform3/LConn1 -- Rigid Transform24/LConn1
  Weld Joint3/RConn1 -- Rigid Transform11/LConn1 -- ColumnLB1/RConn1 -- Weld Joint15/RConn1
  ColumnLB3/LConn1 -- Weld Joint4/LConn1 -- Rigid Transform25/LConn1 -- Rigid Transform12/LConn1
  Weld Joint1/LConn1 -- Rigid Transform1/LConn1 -- ColumnRF1/RConn1 -- Weld Joint12/LConn1
  ColumnRF3/LConn1 -- Weld Joint6/RConn1 -- Rigid Transform17/LConn1 -- Rigid Transform5/LConn1
  Weld Joint2/RConn1 -- Rigid Transform10/LConn1 -- Weld Joint13/LConn1 -- ColumnLF1/RConn1
  ColumnRB3/RConn1 -- Weld Joint8/LConn1
  Weld Joint9/LConn1 -- ColumnRF3/RConn1
  ColumnLB3/RConn1 -- Weld Joint10/RConn1
  Bridging Girder6/RConn1 -- Rigid Transform15/RConn1
  Rigid Transform/RConn1 -- Bridging Girder/LConn1
  Rigid Transform1/RConn1 -- Bridging Girder/RConn1
  Rigid Transform2/RConn1 -- ColumnRB1/LConn1
  RB/RConn1 -- Rigid Transform2/LConn1
  Rigid Transform4/LConn1 -- RF/RConn1
  Rigid Transform4/RConn1 -- RFColMove/RConn1 -- ColumnRF1/LConn1
  Rigid Transform3/RConn1 -- Bridging Girder2/LConn1
  Rigid Transform5/RConn1 -- Bridging Girder2/RConn1
  Rigid Transform6/RConn1 -- Bridging Girder3/LConn1
  Rigid Transform7/RConn1 -- Bridging Girder3/RConn1
  Rigid Transform/LConn1 -- Weld Joint/LConn1 -- ColumnRB1/RConn1 -- Weld Joint14/RConn1
  ColumnRF2/LConn1 -- Weld Joint1/RConn1
  Weld Joint6/LConn1 -- ColumnRF2/RConn1
  Weld Joint7/LConn1 -- ColumnRB2/RConn1
  Rigid Transform6/LConn1 -- Rigid Transform22/LConn1 -- Weld Joint8/RConn1
  Rigid Transform7/LConn1 -- Rigid Transform18/LConn1 -- Weld Joint9/RConn1
  Bridging Girder4/RConn1 -- Rigid Transform10/RConn1
  ColumnLF2/LConn1 -- Weld Joint2/LConn1
  ColumnLB2/LConn1 -- Weld Joint3/LConn1
  Weld Joint4/RConn1 -- ColumnLB2/RConn1
  Weld Joint5/RConn1 -- ColumnLF2/RConn1
  Bridging Girder5/LConn1 -- Rigid Transform12/RConn1
  Rigid Transform14/RConn1 -- Bridging Girder6/LConn1
  Weld Joint11/RConn1 -- ColumnLF3/RConn1
  Weld Joint10/LConn1 -- Rigid Transform23/LConn1 -- Rigid Transform14/LConn1
  Rigid Transform21/LConn1 -- Weld Joint17/RConn1
  Girder1/LConn1 -- Rigid Transform28/LConn1 -- Girder2/RConn1
  Girder2/LConn1 -- Girder3/RConn1 -- Weld Joint19/RConn1
  Rigid Transform16/LConn1 -- Weld Joint12/RConn1
  Rigid Transform19/LConn1 -- Weld Joint13/RConn1
  Rigid Transform16/RConn1 -- Rigid Transform67/RConn1 -- Girder1/RConn1
  LB/RConn1 -- Rigid Transform8/LConn1
  Rigid Transform8/RConn1 -- ColumnLB1/LConn1
  Rigid Transform9/LConn1 -- LF/RConn1
  Rigid Transform9/RConn1 -- LFColMove/RConn1 -- ColumnLF1/LConn1
  Bridging Girder5/RConn1 -- Rigid Transform13/RConn1
  Rigid Transform11/RConn1 -- Bridging Girder4/LConn1
  Rigid Transform17/RConn1 -- Rigid Transform73/RConn1 -- Girder4/RConn1
  Girder5/LConn1 -- Weld Joint18/RConn1 -- Girder6/RConn1
  Girder4/LConn1 -- Weld Joint22/RConn1 -- Girder5/RConn1
  Brick Solid2/LConn1 -- Rigid Transform44/RConn1
  Girder8/LConn1 -- Girder9/RConn1 -- Weld Joint24/RConn1
  Rigid Transform18/RConn1 -- Rigid Transform75/RConn1 -- Girder7/RConn1
  Girder3/LConn1 -- Rigid Transform66/LConn1 -- Rigid Transform19/RConn1
  Girder6/LConn1 -- Rigid Transform72/LConn1 -- Rigid Transform20/RConn1
  Girder9/LConn1 -- Rigid Transform74/LConn1 -- Rigid Transform21/RConn1
  Rigid Transform22/RConn1 -- " LeftFront"/LConn1 -- Girder10/RConn1 -- Rigid Transform76/RConn1
  Girder12/LConn1 -- Rigid Transform77/LConn1 -- Rigid Transform23/RConn1
  Girder11/LConn1 -- 3rdFloorMove/RConn1 -- Rigid Transform50/LConn1 -- Girder12/RConn1
  Girder10/LConn1 -- " LeftFront"/RConn1 -- External Force and Torque2/RConn1 -- Girder11/RConn1 -- Weld Joint25/LConn1
  Girder15/LConn1 -- Rigid Transform70/LConn1 -- Rigid Transform25/RConn1
  Rigid Transform24/RConn1 -- Rigid Transform71/RConn1 -- Girder13/RConn1
  Girder13/LConn1 -- Weld Joint21/LConn1 -- Girder14/RConn1
  Girder14/LConn1 -- Girder15/RConn1 -- Rigid Transform42/LConn1
  Girder18/LConn1 -- Rigid Transform68/LConn1 -- Rigid Transform27/RConn1
  Rigid Transform26/RConn1 -- Girder16/RConn1 -- Rigid Transform69/RConn1
  Brick Solid/LConn2 -- Rigid Transform31/RConn1
  Girder17/LConn1 -- Rigid Transform34/LConn1 -- Girder18/RConn1
  Rigid Transform26/LConn1 -- Weld Joint14/LConn1
  Rigid Transform27/LConn1 -- Weld Joint15/LConn1
  ColumnLF3/LConn1 -- Weld Joint16/LConn1 -- Weld Joint5/LConn1 -- Rigid Transform13/LConn1
  Weld Joint16/RConn1 -- Rigid Transform20/LConn1
  Rigid Transform15/LConn1 -- Weld Joint17/LConn1 -- Weld Joint11/LConn1
  Rigid Transform29/LConn1 -- Rigid Transform28/RConn1
  Brick Solid/LConn1 -- Rigid Transform29/RConn1
  Rigid Transform33/LConn1 -- Rigid Transform32/RConn1
  Brick Solid/RConn1 -- Rigid Transform33/RConn1
  Rigid Transform32/LConn1 -- Weld Joint19/LConn1
  Girder16/LConn1 -- Girder17/RConn1 -- Weld Joint20/LConn1
  Rigid Transform31/LConn1 -- Rigid Transform30/RConn1
  Brick Solid/RConn2 -- Rigid Transform35/RConn1
  Rigid Transform35/LConn1 -- Rigid Transform34/RConn1
  Rigid Transform30/LConn1 -- Weld Joint20/RConn1
  Brick Solid1/RConn1 -- Rigid Transform37/RConn1
  Rigid Transform37/LConn1 -- Rigid Transform36/RConn1
  Rigid Transform36/LConn1 -- Weld Joint18/LConn1
  Brick Solid1/LConn1 -- Rigid Transform38/RConn1
  Rigid Transform38/LConn1 -- Rigid Transform39/RConn1
  Rigid Transform41/LConn1 -- Rigid Transform40/RConn1
  Rigid Transform40/LConn1 -- Weld Joint21/RConn1
  Brick Solid1/LConn2 -- Rigid Transform41/RConn1
  Rigid Transform43/LConn1 -- Rigid Transform42/RConn1
  Brick Solid1/RConn2 -- Rigid Transform43/RConn1
  Rigid Transform39/LConn1 -- Weld Joint22/LConn1
  Weld Joint23/RConn1 -- Girder7/LConn1 -- Girder8/RConn1
  Rigid Transform44/LConn1 -- Rigid Transform45/RConn1
  Rigid Transform45/LConn1 -- Weld Joint23/LConn1
  Rigid Transform47/LConn1 -- Rigid Transform46/RConn1
  Rigid Transform46/LConn1 -- Weld Joint24/LConn1
  Brick Solid2/RConn1 -- Rigid Transform47/RConn1
  Rigid Transform48/LConn1 -- Weld Joint25/RConn1
  Rigid Transform49/LConn1 -- Rigid Transform48/RConn1
  Brick Solid2/LConn2 -- Rigid Transform49/RConn1
  Rigid Transform51/LConn1 -- Rigid Transform50/RConn1
  Brick Solid2/RConn2 -- Rigid Transform51/RConn1
  Simulink-PS Converter6/RConn1 -- External Force and Torque2/LConn6
  External Force and Torque2/LConn3 -- Simulink-PS Converter10/RConn1
  External Force and Torque2/LConn1 -- Simulink-PS Converter2/RConn1
  Simulink-PS Converter5/RConn1 -- External Force and Torque2/LConn5
  Simulink-PS Converter4/RConn1 -- External Force and Torque2/LConn2
  Simulink-PS Converter7/RConn1 -- External Force and Torque2/LConn4
  " LeftFront"/RConn5 -- PS-Simulink Converter19/LConn1
  PS-Simulink Converter5/LConn1 -- " LeftFront"/RConn3
  " LeftFront"/RConn4 -- PS-Simulink Converter1/LConn1
  PS-Simulink Converter6/LConn1 -- " LeftFront"/RConn2
  Rigid Transform52/LConn1 -- ColumnRB1/LConn2
  K bracing/RConn1 -- Rigid Transform53/RConn1
  Rigid Transform56/LConn1 -- Rigid Transform55/RConn1
  K bracing/LConn1 -- Rigid Transform54/RConn1
  Rigid Transform52/RConn1 -- Rigid Transform53/LConn1
  Rigid Transform54/LConn1 -- Rigid Transform59/LConn1 -- Girder17/LConn2
  ColumnLB1/LConn2 -- Rigid Transform57/LConn1
  Rigid Transform58/LConn1 -- Rigid Transform57/RConn1
  K bracing1/LConn1 -- Rigid Transform58/RConn1
  Rigid Transform59/RConn1 -- K bracing1/RConn1
  ColumnRF1/LConn2 -- Weld Joint26/LConn1
  Rigid Transform61/LConn1 -- Rigid Transform60/RConn1
  K bracing2/RConn1 -- Rigid Transform61/RConn1
  K bracing2/LConn1 -- Rigid Transform62/RConn1
  Rigid Transform62/LConn1 -- Rigid Transform65/LConn1 -- Girder2/LConn2
  Weld Joint26/RConn1 -- Rigid Transform60/LConn1
  ColumnLF1/LConn2 -- Weld Joint27/LConn1
  Rigid Transform63/RConn1 -- Rigid Transform64/LConn1
  K bracing3/LConn1 -- Rigid Transform64/RConn1
  Rigid Transform65/RConn1 -- K bracing3/RConn1
  Weld Joint27/RConn1 -- Rigid Transform63/LConn1
  RFColMove/RConn2 -- PS-Simulink Converter2/LConn1
  PS-Simulink Converter3/LConn1 -- RFColMove/RConn3
  PS-Simulink Converter4/LConn1 -- RFColMove/RConn4
  RFColMove/LConn1 -- 3rdFloorMove/LConn1 -- GroundSurface/RConn1 -- LFColMove/LConn1
  PS-Simulink Converter8/LConn1 -- LFColMove/RConn3
  PS-Simulink Converter9/LConn1 -- LFColMove/RConn4
  LFColMove/RConn2 -- PS-Simulink Converter7/LConn1
  PS-Simulink Converter11/LConn1 -- 3rdFloorMove/RConn3
  PS-Simulink Converter12/LConn1 -- 3rdFloorMove/RConn4
  3rdFloorMove/RConn2 -- PS-Simulink Converter10/LConn1
  Bearing Joint1/RConn1 -- Rigid Transform67/LConn1
  Bearing Joint1/LConn1 -- Rigid Transform66/RConn1
  Bearing Joint/LConn1 -- Rigid Transform68/RConn1
  Bearing Joint/RConn1 -- Rigid Transform69/LConn1
  Bearing Joint2/LConn1 -- Rigid Transform70/RConn1
  Bearing Joint2/RConn1 -- Rigid Transform71/LConn1
  Bearing Joint3/RConn1 -- Rigid Transform73/LConn1
  Bearing Joint3/LConn1 -- Rigid Transform72/RConn1
  Bearing Joint4/LConn1 -- Rigid Transform74/RConn1
  Rigid Transform75/LConn1 -- Bearing Joint4/RConn1
  Rigid Transform76/LConn1 -- Bearing Joint5/RConn1
  Bearing Joint5/LConn1 -- Rigid Transform77/RConn1
